simulink model "SWC_FDC_type"  (R2021b)
settings: Solver=FixedStepDiscrete  StartTime=0.0  StopTime=10.0  FixedStep=0.001  RelTol=1e-3
values from neighbouring files (symbols this model uses):
  C_TASK_5MS_S = (	C_TICK_TIME_S      	)    [vcu_local_hdr.m]
  DID_VCUKey = uint16(0x0202)    [vcu_local_hdr.m]
  DID_XWD = uint16(513)    [vcu_local_hdr.m]
  DIDLen_DKCKey = uint16(8)    [vcu_local_hdr.m]
  DIDLen_FoxPiBattSta = uint16(4)    [vcu_local_hdr.m]
  DIDLen_FoxPiBrakeSta = uint16(13)    [vcu_local_hdr.m]
  DIDLen_FoxPiButtonSta = uint16(2)    [vcu_local_hdr.m]
  DIDLen_FoxPiCtrlEnSw = uint16(1)    [vcu_local_hdr.m]
  DIDLen_FoxPiDrivingCtrl = uint16(21)    [vcu_local_hdr.m]
  DIDLen_FoxPiEPSSta = uint16(11)    [vcu_local_hdr.m]
  DIDLen_FoxPiLampCtrl = uint16(6)    [vcu_local_hdr.m]
  DIDLen_FoxPiLampSta = uint16(2)    [vcu_local_hdr.m]
  DIDLen_FoxPiMotionSta = uint16(13)    [vcu_local_hdr.m]
  DIDLen_FoxPiMotorSta = uint16(11)    [vcu_local_hdr.m]
  DIDLen_FoxPiPedalPos = uint16(3)    [vcu_local_hdr.m]
  DIDLen_FoxPiPTGUSSSw = uint16(1)    [vcu_local_hdr.m]
  DIDLen_FoxPiShifterAllow = uint16(3)    [vcu_local_hdr.m]
  DIDLen_FoxPiSwSta = uint16(2)    [vcu_local_hdr.m]
  DIDLen_FoxPiTPMSSta = uint16(13)    [vcu_local_hdr.m]
  DIDLen_FoxPiUSSDist = uint16(20)    [vcu_local_hdr.m]
  DIDLen_FoxPiUSSFaultSta = uint16(2)    [vcu_local_hdr.m]
  DIDLen_FoxPiWheelSpd = uint16(16)    [vcu_local_hdr.m]
  DIDNum_DKCKey = uint16(0x0202)    [vcu_local_hdr.m]
  DIDNum_FoxPiBattSta = uint16(0x100D)    [vcu_local_hdr.m]
  DIDNum_FoxPiBrakeSta = uint16(0x1003)    [vcu_local_hdr.m]
  DIDNum_FoxPiButtonSta = uint16(0x1006)    [vcu_local_hdr.m]
  DIDNum_FoxPiCtrlEnSw = uint16(0x1012)    [vcu_local_hdr.m]
  DIDNum_FoxPiDrivingCtrl = uint16(0x1001)    [vcu_local_hdr.m]
  DIDNum_FoxPiEPSSta = uint16(0x1005)    [vcu_local_hdr.m]
  DIDNum_FoxPiLampCtrl = uint16(0x100C)    [vcu_local_hdr.m]
  DIDNum_FoxPiLampSta = uint16(0x100B)    [vcu_local_hdr.m]
  DIDNum_FoxPiMotionSta = uint16(0x1002)    [vcu_local_hdr.m]
  DIDNum_FoxPiMotorSta = uint16(0x1010)    [vcu_local_hdr.m]
  DIDNum_FoxPiPedalPos = uint16(0x100F)    [vcu_local_hdr.m]
  DIDNum_FoxPiPTGUSSSw = uint16(0x1009)    [vcu_local_hdr.m]
  DIDNum_FoxPiShifterAllow = uint16(0x1011)    [vcu_local_hdr.m]
  DIDNum_FoxPiSwSta = uint16(0x100A)    [vcu_local_hdr.m]
  DIDNum_FoxPiTPMSSta = uint16(0x100E)    [vcu_local_hdr.m]
  DIDNum_FoxPiUSSDist = uint16(0x1007)    [vcu_local_hdr.m]
  DIDNum_FoxPiUSSFaultSta = uint16(0x1008)    [vcu_local_hdr.m]
  DIDNum_FoxPiWheelSpd = uint16(0x1004)    [vcu_local_hdr.m]
  DIDVCUKeyLength = uint16(8)    [vcu_local_hdr.m]
  DTC_10020B = Simulink.Parameter    [DTC_Constant_Definition.m]
  DTC_10020C = Simulink.Parameter    [DTC_Constant_Definition.m]
  DTC_10020D = Simulink.Parameter    [DTC_Constant_Definition.m]
  DTC_10020E = Simulink.Parameter    [DTC_Constant_Definition.m]
  DTC_100210 = Simulink.Parameter    [DTC_Constant_Definition.m]
  DTC_100211 = Simulink.Parameter    [DTC_Constant_Definition.m]
  DTC_100212 = Simulink.Parameter    [DTC_Constant_Definition.m]
  DTC_100213 = Simulink.Parameter    [DTC_Constant_Definition.m]
  DTC_100214 = Simulink.Parameter    [DTC_Constant_Definition.m]
  DTC_100215 = Simulink.Parameter    [DTC_Constant_Definition.m]
  DTC_100216 = Simulink.Parameter    [DTC_Constant_Definition.m]
  DTC_100217 = Simulink.Parameter    [DTC_Constant_Definition.m]
  DTC_100218 = Simulink.Parameter    [DTC_Constant_Definition.m]
  DTC_100219 = Simulink.Parameter    [DTC_Constant_Definition.m]
  DTC_10021A = Simulink.Parameter    [DTC_Constant_Definition.m]
  DTC_10021B = Simulink.Parameter    [DTC_Constant_Definition.m]
  DTC_10021C = Simulink.Parameter    [DTC_Constant_Definition.m]
  DTC_10021D = Simulink.Parameter    [DTC_Constant_Definition.m]
  DTC_10021E = Simulink.Parameter    [DTC_Constant_Definition.m]
  DTC_100220 = Simulink.Parameter    [DTC_Constant_Definition.m]
  DTC_100221 = Simulink.Parameter    [DTC_Constant_Definition.m]
  DTC_100223 = Simulink.Parameter    [DTC_Constant_Definition.m]
  DTC_100224 = Simulink.Parameter    [DTC_Constant_Definition.m]
  DTC_100225 = Simulink.Parameter    [DTC_Constant_Definition.m]
  DTC_100226 = Simulink.Parameter    [DTC_Constant_Definition.m]
  DTC_100227 = Simulink.Parameter    [DTC_Constant_Definition.m]
  DTC_100242 = Simulink.Parameter    [DTC_Constant_Definition.m]
  DTC_100243 = Simulink.Parameter    [DTC_Constant_Definition.m]
  DTC_100244 = Simulink.Parameter    [DTC_Constant_Definition.m]
  DTC_100247 = Simulink.Parameter    [DTC_Constant_Definition.m]
  DTC_100248 = Simulink.Parameter    [DTC_Constant_Definition.m]
  DTC_100249 = Simulink.Parameter    [DTC_Constant_Definition.m]
  DTC_100250 = Simulink.Parameter    [DTC_Constant_Definition.m]
  DTC_100251 = Simulink.Parameter    [DTC_Constant_Definition.m]
  DTC_100252 = Simulink.Parameter    [DTC_Constant_Definition.m]
  DTC_100A10 = Simulink.Parameter    [DTC_Constant_Definition.m]
  DTC_100A12 = Simulink.Parameter    [DTC_Constant_Definition.m]
  DTC_100A16 = Simulink.Parameter    [DTC_Constant_Definition.m]
  DTC_100A17 = Simulink.Parameter    [DTC_Constant_Definition.m]
  DTC_100A18 = Simulink.Parameter    [DTC_Constant_Definition.m]
  DTC_100A19 = Simulink.Parameter    [DTC_Constant_Definition.m]
  DTC_500B01 = Simulink.Parameter    [DTC_Constant_Definition.m]
  DTC_500B02 = Simulink.Parameter    [DTC_Constant_Definition.m]
  DTC_500B03 = Simulink.Parameter    [DTC_Constant_Definition.m]
  DTC_500B04 = Simulink.Parameter    [DTC_Constant_Definition.m]
  DTC_500B05 = Simulink.Parameter    [DTC_Constant_Definition.m]
  DTC_500B06 = Simulink.Parameter    [DTC_Constant_Definition.m]
  DTC_500B07 = Simulink.Parameter    [DTC_Constant_Definition.m]
  DTC_500B08 = Simulink.Parameter    [DTC_Constant_Definition.m]
  DTC_500B09 = Simulink.Parameter    [DTC_Constant_Definition.m]
  DTC_500B0A = Simulink.Parameter    [DTC_Constant_Definition.m]
  DTC_500B0B = Simulink.Parameter    [DTC_Constant_Definition.m]
  DTC_500B0C = Simulink.Parameter    [DTC_Constant_Definition.m]
  DTC_500B0D = Simulink.Parameter    [DTC_Constant_Definition.m]
  DTC_500B0E = Simulink.Parameter    [DTC_Constant_Definition.m]
  DTC_500B0F = Simulink.Parameter    [DTC_Constant_Definition.m]
  DTC_500B10 = Simulink.Parameter    [DTC_Constant_Definition.m]
  DTC_90021F = Simulink.Parameter    [DTC_Constant_Definition.m]
  DTC_90022F = Simulink.Parameter    [DTC_Constant_Definition.m]
  DTC_900253 = Simulink.Parameter    [DTC_Constant_Definition.m]
  DTC_900254 = Simulink.Parameter    [DTC_Constant_Definition.m]
  DTC_900301 = Simulink.Parameter    [DTC_Constant_Definition.m]
  DTC_900302 = Simulink.Parameter    [DTC_Constant_Definition.m]
  DTC_900303 = Simulink.Parameter    [DTC_Constant_Definition.m]
  DTC_900304 = Simulink.Parameter    [DTC_Constant_Definition.m]
  DTC_900305 = Simulink.Parameter    [DTC_Constant_Definition.m]
  DTC_900909 = Simulink.Parameter    [DTC_Constant_Definition.m]
  DTC_90090A = Simulink.Parameter    [DTC_Constant_Definition.m]
  DTC_90090B = Simulink.Parameter    [DTC_Constant_Definition.m]
  DTC_90090C = Simulink.Parameter    [DTC_Constant_Definition.m]
  DTC_90090D = Simulink.Parameter    [DTC_Constant_Definition.m]
  DTC_90090E = Simulink.Parameter    [DTC_Constant_Definition.m]
  DTC_90090F = Simulink.Parameter    [DTC_Constant_Definition.m]
  DTC_900910 = Simulink.Parameter    [DTC_Constant_Definition.m]
  DTC_900911 = Simulink.Parameter    [DTC_Constant_Definition.m]
  DTC_900912 = Simulink.Parameter    [DTC_Constant_Definition.m]
  DTC_900913 = Simulink.Parameter    [DTC_Constant_Definition.m]
  DTC_900914 = Simulink.Parameter    [DTC_Constant_Definition.m]
  ... (+54 more)
undefined symbols (not defined in the file or in its folder): f32_ApsOutVehSpdSig, KHAL_CANBusOffDebounce_cnt, KHAL_CANBusOffDebounce_s, KHAL_DKCDecryptEnable_flg_ovrdflg, KHAL_DKCDecryptEnable_flg_ovrdval, KHAL_RandomNumberY1_enum, KHAL_RandomNumberY2_enum, KHAL_RandomNumberY_ovrdflg, KHAL_TPMSRESBUTT_flg_ovrdflg, KHAL_TPMSRESBUTT_flg_ovrdval, KINP_ReadVinCode_flg, P_boolean, R_DIDWriteCDD_CSOP_DIDSet_DKCKey, R_DIDWriteCDD_CSOP_DIDSet_FoxPiBattSta, R_DIDWriteCDD_CSOP_DIDSet_FoxPiBrakeSta, R_DIDWriteCDD_CSOP_DIDSet_FoxPiButtonSta, R_DIDWriteCDD_CSOP_DIDSet_FoxPiCtrlEnSw, R_DIDWriteCDD_CSOP_DIDSet_FoxPiDrivingCtrl, R_DIDWriteCDD_CSOP_DIDSet_FoxPiEPSSta, R_DIDWriteCDD_CSOP_DIDSet_FoxPiLampCtrl, R_DIDWriteCDD_CSOP_DIDSet_FoxPiLampSta, R_DIDWriteCDD_CSOP_DIDSet_FoxPiMotionSta, R_DIDWriteCDD_CSOP_DIDSet_FoxPiMotorSta, R_DIDWriteCDD_CSOP_DIDSet_FoxPiPedalPos, R_DIDWriteCDD_CSOP_DIDSet_FoxPiPTGUSSSw, R_DIDWriteCDD_CSOP_DIDSet_FoxPiShifterAllow, R_DIDWriteCDD_CSOP_DIDSet_FoxPiSwSta, R_DIDWriteCDD_CSOP_DIDSet_FoxPiTPMSSta, R_DIDWriteCDD_CSOP_DIDSet_FoxPiUSSDist, R_DIDWriteCDD_CSOP_DIDSet_FoxPiUSSFaultSta, R_DIDWriteCDD_CSOP_DIDSet_FoxPiWheelSpd, R_E2E_CAN3_VCU1_CSOP_Write_CAN3_VCU1, R_E2E_CAN3_VCU1_toNIDEC_CSOP_Write_CAN3_VCU1_toNIDEC, R_E2E_CAN4_VCU1_CSOP_Write_CAN4_VCU1, R_FDCCDD_Inner_CSOP_FDC_AppCallSleep, R_HALIN_IMU_CSOP_IMUSetSta, R_HALINCDD_CSOP_PAS_Handler, R_HALINCDD_CSOP_ResetPedalZeroPosDone, R_HALINCDD_CSOP_TPMSSensorIDRegSetResults, R_HALINCDD_CSOP_UDS_Main, R_HALOUT_APS_CSOP_ApsOutput, R_HALOUTCDD_CSOP_AppNmStateReq, R_HALOUTCDD_CSOP_IVIReset, R_HALOUTCDD_CSOP_SetAcoreRebootCmdACK, R_HALOUTCDD_CSOP_SetSysPwrStat ... (+80)
libraries: FVT_lib x447, simulink x289, hcu_lib x19, hdlsllib x9, app x1, halin x1, halout x1, matrix_library x1, inp x1, outp x1
(part 9 of 15)

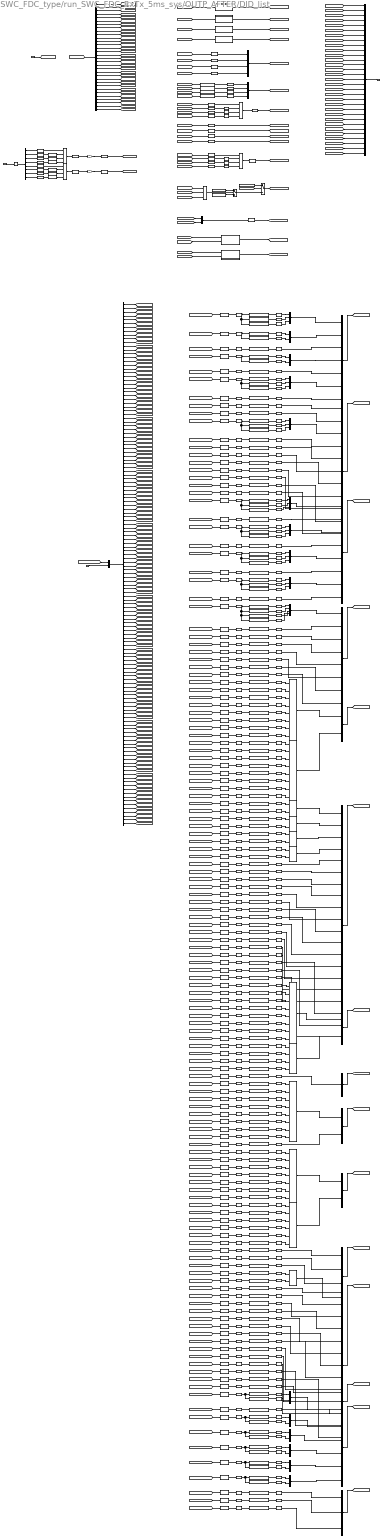
== system SWC_FDC_type/run_SWC_FDC_RxTx_5ms_sys/OUTP_AFTER/DID_list ==
  BOUTP_outputs : Inport
  VHAL_NvmReadArray_raw : Inport  Port=2
  BINP_CANx_outputs : Inport  Port=3
  Bit Shift : hdlsllib/Logic and Bit Operations/Bit Shift  mode=Shift Left Logical  N=3
  Bit Shift1 : hdlsllib/Logic and Bit Operations/Bit Shift  mode=Shift Left Logical  N=2
  Bit Shift2 : hdlsllib/Logic and Bit Operations/Bit Shift  mode=Shift Left Logical  N=1
  Bit Shift3 : hdlsllib/Logic and Bit Operations/Bit Shift  mode=Shift Left Logical  N=3
  Bit Shift4 : hdlsllib/Logic and Bit Operations/Bit Shift  mode=Shift Left Logical  N=2
  Bit Shift5 : hdlsllib/Logic and Bit Operations/Bit Shift  mode=Shift Left Logical  N=1
  Bitwise OR : simulink/Logic and Bit Operations/Bitwise Operator  logicop=OR  UseBitMask=off  NumInputPorts=4  BitMask=bin2dec('11011001')  BitMaskRealWorld=Stored Integer
  Bitwise OR1 : simulink/Logic and Bit Operations/Bitwise Operator  logicop=OR  UseBitMask=off  NumInputPorts=4  BitMask=bin2dec('11011001')  BitMaskRealWorld=Stored Integer
  Bitwise OR13 : simulink/Logic and Bit Operations/Bitwise Operator  logicop=OR  UseBitMask=off  NumInputPorts=4  BitMask=bin2dec('00000000000000000000')  BitMaskRealWorld=Stored Integer
  Bitwise OR14 : simulink/Logic and Bit Operations/Bitwise Operator  logicop=OR  UseBitMask=off  NumInputPorts=4  BitMask=bin2dec('00000000000000000000')  BitMaskRealWorld=Stored Integer
  BitwiseAND{,1,6,8} (4 alike) : simulink/Logic and Bit Operations/Bitwise Operator  logicop=OR  UseBitMask=off  NumInputPorts=8  BitMask=bin2dec('11011001')  BitMaskRealWorld=Stored Integer
  BitwiseAND10 : simulink/Logic and Bit Operations/Bitwise Operator  logicop=OR  UseBitMask=off  NumInputPorts=6  BitMask=bin2dec('11011001')  BitMaskRealWorld=Stored Integer
  BitwiseAND{2..5,11} (5 alike) : simulink/Logic and Bit Operations/Bitwise Operator  logicop=OR  UseBitMask=off  NumInputPorts=2  BitMask=bin2dec('11011001')  BitMaskRealWorld=Stored Integer
  BitwiseAND7 : simulink/Logic and Bit Operations/Bitwise Operator  logicop=OR  UseBitMask=off  NumInputPorts=4  BitMask=bin2dec('11011001')  BitMaskRealWorld=Stored Integer
  BitwiseAND9 : simulink/Logic and Bit Operations/Bitwise Operator  logicop=OR  UseBitMask=off  NumInputPorts=7  BitMask=bin2dec('11011001')  BitMaskRealWorld=Stored Integer
  Bus Creator : BusCreator  Inputs=31
  Bus Creator1 : BusCreator  Inputs=2
  Bus Selector : BusSelector  OutputSignals=VOUTP_WriteChkLFID_raw,VOUTP_WriteChkRFID_raw,VOUTP_WriteChkLRID_raw,VOUTP_WriteChkRRID_raw,VOUTP_LFWheelPress_raw8,VOUTP_RFWheelPress_raw8,VOUTP_LRWheelPress_raw8,VOUTP_RRWheelPress_raw8,VOUTP_LFWheelTemp_C,VOUTP_RFWheelTemp_C,VOUTP_LRWheelTemp_C,VOUTP_RRWheelTemp_C,VOUTP_LFBatWarn_flg,VOUTP_RFBatWarn_flg,VOUTP_LRBatWarn_flg,VOUTP_RRBatWarn_flg,VOUTP_LFWheelPSW_raw8,VOUTP_LRWheelPSW_raw8,VOUTP_RFWheelPSW_raw8,VOUTP_RRWheelPSW_raw8,VOUTP_LFSensorMode_flg,VOUTP_RFSensorMode_flg,VOUTP_LRSensorMode_flg,VOUTP_RRSensorMode_flg,VOUTP_ALFin_flg,VOUTP_ChkStorge_flg,VOUTP_TPMSStorge_flg,VOUTP_unlearnSfali_flg,VOUTP_WritingCnt_enum,VOUTP_LProgress_enum,VOUTP_EAPS1MIN_pct,VOUTP_EAPS2MIN_pct
  Constant : Constant  Value=ENUM_TPMSLearnStatus_LEARNFAIL
  Constant1 : Constant  Value=ENUM_TPMSLearnStatus_NOTLEARN
  Constant2 : Constant  Value=ENUM_TPMSLearnStatus_LEARNED
  Data Type Conversion{1..23} (23 alike) : DataTypeConversion  OutDataTypeStr=uint8
  Data Type Conversion168 : DataTypeConversion  OutDataTypeStr=single
  Data Type Conversion{169..178} (10 alike) : DataTypeConversion  OutDataTypeStr=uint32
  Data Type Conversion179 : DataTypeConversion  OutDataTypeStr=single
  Demux : Demux  Outputs=8
  Logical Operator1 : Logic  Operator=OR  Inputs=3  AllPortsSameDT=off  OutDataTypeStr=boolean
  Multiply1 : Gain  Gain=1/10000
  Multiply2 : Gain  Gain=1/10000
  Mux{,2,12,20} (4 alike) : Mux
  Mux{1,4..5,14,16,18..19,22..28} (14 alike) : Mux  Inputs=2
  Mux{3,6,8,10,30..33} (8 alike) : Mux  Inputs=3
  Mux11 : Mux  Inputs=8
  Mux13 : Mux  Inputs=8
  Mux15 : Mux  Inputs=20
  Mux17 : Mux  Inputs=1
  Mux21 : Mux  Inputs=13
  Mux29 : Mux  Inputs=6
  Mux7 : Mux  Inputs=7
  Mux9 : Mux  Inputs=11
  Selector1 : Selector  InputPortWidth=256  IndexOptions=Index vector (dialog)  Indices=[112:119]  OutputSizes=1
  Shift Arithmetic37 : ArithShift  BitShiftNumber=8  BitShiftDirection=Left
  Shift Arithmetic38 : ArithShift  BitShiftNumber=16  BitShiftDirection=Left
  Shift Arithmetic39 : ArithShift  BitShiftNumber=24  BitShiftDirection=Left
  Shift Arithmetic40 : ArithShift  BitShiftNumber=8  BitShiftDirection=Left
  Shift Arithmetic41 : ArithShift  BitShiftNumber=16  BitShiftDirection=Left
  Shift Arithmetic42 : ArithShift  BitShiftNumber=24  BitShiftDirection=Left
  SignalPack{,9,15,26,30,34,38,43} (8 alike) : FVT_lib/hal/SignalPack_shiftAfterMask  RightShiftCnt=16  BitMask=16711680  LeftShiftCnt=0
  SignalPack{1,3,6,10,16,27,31,35,39,44,147,150,152,154,156,158} (16 alike) : FVT_lib/hal/SignalPack_shiftAfterMask  RightShiftCnt=8  BitMask=65280  LeftShiftCnt=0
  SignalPack{60,68,100,113,121,132} (6 alike) : FVT_lib/hal/SignalPack_shiftAfterMask  RightShiftCnt=0  BitMask=2^1-1  LeftShiftCnt=7
  SignalPack{53,61,92..93,101,105..106,114,122} (9 alike) : FVT_lib/hal/SignalPack_shiftAfterMask  RightShiftCnt=0  BitMask=2^1-1  LeftShiftCnt=0
  SignalPack{54,62,94,102,107,123} (6 alike) : FVT_lib/hal/SignalPack_shiftAfterMask  RightShiftCnt=0  BitMask=2^1-1  LeftShiftCnt=1
  SignalPack{55,63,95,103,108,116,124} (7 alike) : FVT_lib/hal/SignalPack_shiftAfterMask  RightShiftCnt=0  BitMask=2^1-1  LeftShiftCnt=2
  SignalPack{56,64,96,104,109,117,125} (7 alike) : FVT_lib/hal/SignalPack_shiftAfterMask  RightShiftCnt=0  BitMask=2^1-1  LeftShiftCnt=3
  SignalPack{2,4,7,11,17,28,32,36,40,45,148,151,153,155,157,159} (16 alike) : FVT_lib/hal/SignalPack_shiftAfterMask  RightShiftCnt=0  BitMask=255  LeftShiftCnt=0
  SignalPack{57,65,97,110,118,126} (6 alike) : FVT_lib/hal/SignalPack_shiftAfterMask  RightShiftCnt=0  BitMask=2^1-1  LeftShiftCnt=4
  SignalPack{58,66,98,111,119,127} (6 alike) : FVT_lib/hal/SignalPack_shiftAfterMask  RightShiftCnt=0  BitMask=2^1-1  LeftShiftCnt=5
  SignalPack{59,67,99,112,120,131} (6 alike) : FVT_lib/hal/SignalPack_shiftAfterMask  RightShiftCnt=0  BitMask=2^1-1  LeftShiftCnt=6
  SignalPack115 : FVT_lib/hal/SignalPack_shiftAfterMask  RightShiftCnt=0  BitMask=2^2-1  LeftShiftCnt=0
  SignalPack{5,8,12..14,18..25,29,33,37,41,46..52,77..88,128..130,133..144,146,149,160..162} (56 alike) : FVT_lib/hal/SignalPack_shiftAfterMask  RightShiftCnt=0  BitMask=2^8-1  LeftShiftCnt=0
  SignalPack145 : FVT_lib/hal/SignalPack_shiftAfterMask  RightShiftCnt=0  BitMask=2^2-1  LeftShiftCnt=0
  SignalPack42 : FVT_lib/hal/SignalPack_shiftAfterMask  RightShiftCnt=24  BitMask=4278190080  LeftShiftCnt=0
  SignalPack{69,71,73,75,90} (5 alike) : FVT_lib/hal/SignalPack_shiftAfterMask  RightShiftCnt=0  BitMask=2^4-1  LeftShiftCnt=0
  SignalPack{70,72,74,76} (4 alike) : FVT_lib/hal/SignalPack_shiftAfterMask  RightShiftCnt=0  BitMask=2^4-1  LeftShiftCnt=4
  SignalPack89 : FVT_lib/hal/SignalPack_shiftAfterMask  RightShiftCnt=0  BitMask=2^3-1  LeftShiftCnt=0
  SignalPack91 : FVT_lib/hal/SignalPack_shiftAfterMask  RightShiftCnt=0  BitMask=2^2-1  LeftShiftCnt=0
  Switch : Switch  Criteria=u2 ~= 0
  Switch1 : Switch  Criteria=u2 ~= 0
  UnitConverter{,14,24,44,50,56,62,68} (8 alike) : DataTypeConversion  OutDataTypeStr=uint32
  UnitConverter{1..3,5..8,10..13,15..23,25..43,45..49,51..55,57..61,63..67,69..274,276..279,281..282,284..285,287..288,290..291,293..300} (285 alike) : DataTypeConversion  OutDataTypeStr=uint8
  UnitConverter{4,9,275,280,283,286,289,292} (8 alike) : DataTypeConversion  OutDataTypeStr=uint16
  bus_selector : BusSelector  OutputSignals=BINP_CANx_outputs.BINP_CAN1_outputs.VINP_VehSpeed_kph,BINP_CANx_outputs.BINP_CAN1_outputs.VINP_LongAccel_Gps,BINP_CANx_outputs.BINP_CAN1_outputs.VINP_LongAccelV_flg,BINP_CANx_outputs.BINP_CAN1_outputs.VINP_LatAccel_Gps,BINP_CANx_outputs.BINP_CAN1_outputs.VINP_LatAccelV_flg,BINP_CANx_outputs.BINP_CAN1_outputs.VINP_YawRate_degps,BINP_CANx_outputs.BINP_CAN1_outputs.VINP_YawRateV_flg,BINP_CANx_outputs.BINP_CAN1_outputs.VINP_BrkSwSta_flg,BINP_CANx_outputs.BINP_CAN1_outputs.VINP_BrkSwV_flg,BINP_CANx_outputs.BINP_CAN1_outputs.VINP_MCPressure_bar,BINP_CANx_outputs.BINP_CAN1_outputs.VINP_MCPressureV_flg,BINP_CANx_outputs.BINP_CAN1_outputs.VINP_PBAActive_flg,BINP_CANx_outputs.BINP_CAN1_outputs.VINP_PBAFailed_flg,BINP_CANx_outputs.BINP_CAN1_outputs.VINP_ABSActive_flg,BINP_CANx_outputs.BINP_CAN1_outputs.VINP_ABSFailed_flg,BINP_CANx_outputs.BINP_CAN1_outputs.VINP_EBDActive_flg,BINP_CANx_outputs.BINP_CAN1_outputs.VINP_EBDFailed_flg,BINP_CANx_outputs.BINP_CAN1_outputs.VINP_ACCAvail_flg,BINP_CANx_outputs.BINP_CAN1_outputs.VINP_RRRawWhlSpeed_kph,BINP_CANx_outputs.BINP_CAN1_outputs.VINP_RRRawWhlSpeedV_flg,BINP_CANx_outputs.BINP_CAN1_outputs.VINP_LRRawWhlSpeed_kph,BINP_CANx_outputs.BINP_CAN1_outputs.VINP_LRRawWhlSpeedV_flg,BINP_CANx_outputs.BINP_CAN1_outputs.VINP_RFRawWhlSpeed_kph,BINP_CANx_outputs.BINP_CAN1_outputs.VINP_RFRawWhlSpeedV_flg,BINP_CANx_outputs.BINP_CAN1_outputs.VINP_LFRawWhlSpeed_kph,BINP_CANx_outputs.BINP_CAN1_outputs.VINP_LFRawWhlSpeedV_flg,BINP_CANx_outputs.BINP_CAN1_outputs.VINP_SASAngle_Deg,BINP_CANx_outputs.BINP_CAN1_outputs.VINP_SASV_flg,BINP_CANx_outputs.BINP_CAN1_outputs.VINP_SASCAL_flg,BINP_CANx_outputs.BINP_CAN1_outputs.VINP_EPSAOIControl_enum,BINP_CANx_outputs.BINP_CAN1_outputs.VINP_EpasFailed_enum,BINP_CANx_outputs.BINP_CAN1_outputs.VINP_EPSTOIActivation_flg,BINP_CANx_outputs.BINP_CAN1_outputs.VINP_EPSTOIUnavailable_flg,BINP_CANx_outputs.BINP_CAN1_outputs.VINP_EPSTOIFault_flg,BINP_CANx_outputs.BINP_CAN4_outputs.VINP_SWCACCSta_flg,BINP_CANx_outputs.BINP_CAN4_outputs.VINP_SWCCANCELSta_flg,BINP_CANx_outputs.BINP_CAN4_outputs.VINP_SWCSetdownSta_flg,BINP_CANx_outputs.BINP_CAN4_outputs.VINP_SWCResUpSta_flg,BINP_CANx_outputs.BINP_CAN4_outputs.VINP_SWCDistanceSta_flg,BINP_CANx_outputs.BINP_CAN4_outputs.VINP_SWCmodeSta_flg,BINP_CANx_outputs.BINP_CAN4_outputs.VINP_SWCUpSta_flg,BINP_CANx_outputs.BINP_CAN4_outputs.VINP_SWCDownSta_flg,BINP_CANx_outputs.BINP_CAN4_outputs.VINP_SWCLeftSta_flg,BINP_CANx_outputs.BINP_CAN4_outputs.VINP_SWCRightSta_flg,BINP_CANx_outputs.BINP_CAN4_outputs.VINP_SWCRegenDown_flg,BINP_CANx_outputs.BINP_CAN4_outputs.VINP_SWCUndefinedSta_flg,BINP_CANx_outputs.BINP_CAN4_outputs.VINP_SWCVRSta_flg,BINP_CANx_outputs.BINP_CAN4_outputs.VINP_SWCLKASta_flg,BINP_CANx_outputs.BINP_CAN4_outputs.VINP_SWCRegenUp_flg,BINP_CANx_outputs.BINP_CAN4_outputs.VINP_SWCTripSta_flg,BOUTP_outputs.VOUTP_PASARMR_enum,BOUTP_outputs.VOUTP_PASARML_enum,BOUTP_outputs.VOUTP_PASARCR_enum,BOUTP_outputs.VOUTP_PASARCL_enum,BOUTP_outputs.VOUTP_PASAFMR_enum,BOUTP_outputs.VOUTP_PASAFML_enum,BOUTP_outputs.VOUTP_PASAFCR_enum,BOUTP_outputs.VOUTP_PASAFCL_enum,BOUTP_outputs.VOUTP_PASDRMR_cm,BOUTP_outputs.VOUTP_PASDRML_cm,BOUTP_outputs.VOUTP_PASDRCR_cm,BOUTP_outputs.VOUTP_PASDRCL_cm,BOUTP_outputs.VOUTP_PASDFMR_cm,BOUTP_outputs.VOUTP_PASDFML_cm,BOUTP_outputs.VOUTP_PASDFCR_cm,BOUTP_outputs.VOUTP_PASDFCL_cm,BOUTP_outputs.VOUTP_APSDFLL_cm,BOUTP_outputs.VOUTP_APSDFLR_cm,BOUTP_outputs.VOUTP_APSDRLL_cm,BOUTP_outputs.VOUTP_APSDRLR_cm,BOUTP_outputs.VOUTP_Chime_enum,BOUTP_outputs.VOUTP_SNSRLayout_enum,BOUTP_outputs.VOUTP_ModOperation_enum,BOUTP_outputs.VOUTP_StaFSya_flg,BOUTP_outputs.VOUTP_USSStaRMR_flg,BOUTP_outputs.VOUTP_USSStaRML_flg,BOUTP_outputs.VOUTP_USSStaRCR_flg,BOUTP_outputs.VOUTP_USSStaRCL_flg,BOUTP_outputs.VOUTP_USSStaFMR_flg,BOUTP_outputs.VOUTP_USSStaFML_flg,BOUTP_outputs.VOUTP_USSStaFCR_flg,BOUTP_outputs.VOUTP_USSStaFCL_flg,BOUTP_outputs.VOUTP_USSStaRLR_flg,BOUTP_outputs.VOUTP_USSStaRLL_flg,BOUTP_outputs.VOUTP_USSStaFLR_flg,BOUTP_outputs.VOUTP_USSStaFLL_flg,BINP_CANx_outputs.BINP_CAN2_outputs.VINP_IVIPTGUSStaSW_flg,BOUTP_outputs.VOUTP_CrashDetd_flg,BINP_CANx_outputs.BINP_CAN4_outputs.VINP_DrLockSta_flg,BOUTP_outputs.VOUTP_AllDoorSW_flg,BOUTP_outputs.VOUTP_DrDoorSW_flg,BOUTP_outputs.VOUTP_PsDoorSW_flg,BOUTP_outputs.VOUTP_RLDoorSW_flg,BOUTP_outputs.VOUTP_RRDoorSW_flg,BOUTP_outputs.VOUTP_TailgateSW_flg,BOUTP_outputs.VOUTP_HoodSW_flg,BOUTP_outputs.VOUTP_TurnSwSta_enum,BOUTP_outputs.VOUTP_DimSwSta_flg,BOUTP_outputs.VOUTP_PassSWSta_flg,BOUTP_outputs.VOUTP_PosLamp_flg,BOUTP_outputs.VOUTP_LBeam_flg,BOUTP_outputs.VOUTP_HBeam_flg,BOUTP_outputs.VOUTP_RDRL_flg,BOUTP_outputs.VOUTP_LDRL_flg,BOUTP_outputs.VOUTP_LTurnLP_flg,BOUTP_outputs.VOUTP_RTurnLP_flg,BOUTP_outputs.VOUTP_BrakeLamp_flg,BOUTP_outputs.VOUTP_ReverseLamp_flg,BOUTP_outputs.VOUTP_RrFogLamp_flg,BINP_CANx_outputs.BINP_CAN3_outputs.VINP_LVBattDet12V_V,BINP_CANx_outputs.BINP_CAN3_outputs.VINP_HVBattSOC_pct,BINP_CANx_outputs.BINP_CAN3_outputs.VINP_CellTempAvg_C,BINP_CANx_outputs.BINP_CAN3_outputs.VINP_HVBContactorSta_flg,BINP_CANx_outputs.BINP_CAN3_outputs.VINP_HVBattErr_flg,BOUTP_outputs.VOUTP_LFWheelPress_raw8,BOUTP_outputs.VOUTP_RFWheelPress_raw8,BOUTP_outputs.VOUTP_LRWheelPress_raw8,BOUTP_outputs.VOUTP_RRWheelPress_raw8,BOUTP_outputs.VOUTP_LFWheelTemp_C,BOUTP_outputs.VOUTP_RFWheelTemp_C,BOUTP_outputs.VOUTP_LRWheelTemp_C,BOUTP_outputs.VOUTP_RRWheelTemp_C,BOUTP_outputs.VOUTP_LFWheelPSW_raw8,BOUTP_outputs.VOUTP_RFWheelPSW_raw8,BOUTP_outputs.VOUTP_LRWheelPSW_raw8,BOUTP_outputs.VOUTP_RRWheelPSW_raw8,BOUTP_outputs.VOUTP_TPMSWarnIndi_enum,BOUTP_outputs.VOUTP_ActAPSPosn_pct,BINP_CANx_outputs.BINP_CAN1_outputs.VINP_BrkPedalPos_pct,BOUTP_outputs.VOUTP_TqSourceRr_enum,BOUTP_outputs.VOUTP_RrTMTqReq_Nm,BINP_CANx_outputs.BINP_CAN3_outputs.VINP_RrEDURealTMTqNidec_Nm,BINP_CANx_outputs.BINP_CAN3_outputs.VINP_RrMotorAvailTqNidec_Nm,BINP_CANx_outputs.BINP_CAN3_outputs.VINP_RrRegenAvailTqNidec_Nm,BINP_CANx_outputs.BINP_CAN3_outputs.VINP_RrTMSpdNidec_rpm,BOUTP_outputs.VOUTP_ExternalTqAllow_flg,BOUTP_outputs.VOUTP_ExtShftAllow_flg,BOUTP_outputs.VOUTP_ExtDoorAllow_flg
  convert_out{,1..3,111,118..121} (9 alike) : FVT_lib/hal/convert_out  gain=1  offset=-40
  convert_out{6,8,10..17,19,21,23,25,27..92,94..108,112..113,126,129,135..141} (106 alike) : FVT_lib/hal/convert_out  gain=1  offset=0
  convert_out109 : FVT_lib/hal/convert_out  gain=0.1  offset=0
  convert_out110 : FVT_lib/hal/convert_out  gain=0.4  offset=0
  convert_out{114..117,122..125} (8 alike) : FVT_lib/hal/convert_out  gain=0.25  offset=7.26
  convert_out127 : FVT_lib/hal/convert_out  gain=0.394  offset=0
  convert_out128 : FVT_lib/hal/convert_out  gain=0.4  offset=0
  convert_out130 : FVT_lib/hal/convert_out  gain=1  offset=-530
  convert_out131 : FVT_lib/hal/convert_out  gain=1  offset=-1023
  convert_out132 : FVT_lib/hal/convert_out  gain=1  offset=-1023
  convert_out133 : FVT_lib/hal/convert_out  gain=1  offset=-1023
  convert_out134 : FVT_lib/hal/convert_out  gain=1  offset=-32767
  convert_out{18,20,22,24} (4 alike) : FVT_lib/hal/convert_out  gain=0.0625  offset=0
  convert_out26 : FVT_lib/hal/convert_out  gain=0.1  offset=-900
  convert_out4 : FVT_lib/hal/convert_out  gain=0.125  offset=0
  convert_out5 : FVT_lib/hal/convert_out  gain=0.01  offset=-1.27
  convert_out7 : FVT_lib/hal/convert_out  gain=0.01  offset=-1.27
  convert_out9 : FVT_lib/hal/convert_out  gain=0.1  offset=-100
  convert_out93 : FVT_lib/hal/convert_out  gain=0.1  offset=-9.7
  pct2raw1 : Subsystem
  pct2raw8 : Subsystem
  uint32Touint8Array : Subsystem
  uint32Touint8Array1 : Subsystem
  uint32Touint8Array2 : Subsystem
  uint32Touint8Array3 : Subsystem
  BOUTP_DIDSetData_outputs : Outport
  wires:
  Bus Selector/1 -> [VOUTP_WriteChkLFID_raw]  "<VOUTP_WriteChkLFID_raw>"
  Bus Selector/2 -> [VOUTP_WriteChkRFID_raw]  "<VOUTP_WriteChkRFID_raw>"
  Bus Selector/4 -> [VOUTP_WriteChkRRID_raw]  "<VOUTP_WriteChkRRID_raw>"
  Bus Selector/3 -> [VOUTP_WriteChkLRID_raw]  "<VOUTP_WriteChkLRID_raw>"
  Bus Selector/5 -> [VOUTP_LFWheelPress_raw8]  "<VOUTP_LFWheelPress_raw8>"
  Bus Selector/6 -> [VOUTP_RFWheelPress_raw8]  "<VOUTP_RFWheelPress_raw8>"
  Bus Selector/7 -> [VOUTP_LRWheelPress_raw8]  "<VOUTP_LRWheelPress_raw8>"
  Bus Selector/8 -> [VOUTP_RRWheelPress_raw8]  "<VOUTP_RRWheelPress_raw8>"
  Bus Selector/13 -> [VOUTP_LFBatWarn_flg]  "<VOUTP_LFBatWarn_flg>"
  Bus Selector/14 -> [VOUTP_RFBatWarn_flg]  "<VOUTP_RFBatWarn_flg>"
  Bus Selector/15 -> [VOUTP_LRBatWarn_flg]  "<VOUTP_LRBatWarn_flg>"
  Bus Selector/16 -> [VOUTP_RRBatWarn_flg]  "<VOUTP_RRBatWarn_flg>"
  Bus Selector/18 -> [VOUTP_LRWheelPSW_raw8]  "<VOUTP_LRWheelPSW_raw8>"
  Bus Selector/19 -> [VOUTP_RFWheelPSW_raw8]  "<VOUTP_RFWheelPSW_raw8>"
  Bus Selector/20 -> [VOUTP_RRWheelPSW_raw8]  "<VOUTP_RRWheelPSW_raw8>"
  Bus Selector/17 -> [VOUTP_LFWheelPSW_raw8]  "<VOUTP_LFWheelPSW_raw8>"
  Bus Selector/21 -> [VOUTP_LFSensorMode_flg]  "<VOUTP_LFSensorMode_flg>"
  Bus Selector/22 -> [VOUTP_RFSensorMode_flg]  "<VOUTP_RFSensorMode_flg>"
  Bus Selector/23 -> [VOUTP_LRSensorMode_flg]  "<VOUTP_LRSensorMode_flg>"
  Bus Selector/24 -> [VOUTP_RRSensorMode_flg]  "<VOUTP_RRSensorMode_flg>"
  Bus Selector/27 -> [VOUTP_TPMSStorge_flg]  "<VOUTP_TPMSStorge_flg>"
  Bus Selector/25 -> [VOUTP_ALFin_flg]  "<VOUTP_ALFin_flg>"
  Bus Selector/26 -> [VOUTP_ChkStorge_flg]  "<VOUTP_ChkStorge_flg>"
  Bus Selector/28 -> [VOUTP_unlearnSfali_flg]  "<VOUTP_unlearnSfali_flg>"
  Bus Selector/9 -> [VOUTP_LFWheelTemp_C]  "<VOUTP_LFWheelTemp_C>"
  Bus Selector/10 -> [VOUTP_RFWheelTemp_C]  "<VOUTP_RFWheelTemp_C>"
  Bus Selector/11 -> [VOUTP_LRWheelTemp_C]  "<VOUTP_LRWheelTemp_C>"
  Bus Selector/12 -> [VOUTP_RRWheelTemp_C]  "<VOUTP_RRWheelTemp_C>"
  Data Type Conversion8/1 -> Mux2/1
  Data Type Conversion9/1 -> Mux2/2
  Data Type Conversion10/1 -> Mux2/3
  Data Type Conversion11/1 -> Mux2/4
  [VOUTP_LFWheelPSW_raw8] -> Data Type Conversion6/1
  [VOUTP_RRWheelPSW_raw8] -> Data Type Conversion5/1
  [VOUTP_LFSensorMode_flg] -> Data Type Conversion21/1
  [VOUTP_RRSensorMode_flg] -> Data Type Conversion14/1
  [VOUTP_LRSensorMode_flg] -> Data Type Conversion12/1
  [VOUTP_RFSensorMode_flg] -> Data Type Conversion13/1
  Data Type Conversion21/1 -> Bitwise OR/1
  Data Type Conversion12/1 -> Bit Shift1/1
  Data Type Conversion14/1 -> Bit Shift/1
  Constant1/1 -> Switch1/3
  [VOUTP_ALFin_flg] -> Logical Operator1/1
  Switch1/1 -> Switch/3
  [VOUTP_ChkStorge_flg] -> Logical Operator1/2
  Constant/1 -> Switch/1
  Constant2/1 -> Switch1/1
  [VOUTP_TPMSStorge_flg] -> Logical Operator1/3
  Logical Operator1/1 -> Switch1/2
  [VOUTP_unlearnSfali_flg] -> Switch/2
  Mux/1 -> [VHAL_DIDSetWhlPres_raw8]
  Mux2/1 -> [VHAL_DIDSetWhlTmp_raw8]
  Data Type Conversion6/1 -> [VHAL_DIDSetLFLowPresThre_raw8]
  Data Type Conversion7/1 -> [VHAL_DIDSetRFLowPresThre_raw8]
  Data Type Conversion4/1 -> [VHAL_DIDSetLRLowPresThre_raw8]
  Data Type Conversion5/1 -> [VHAL_DIDSetRRLowPresThre_raw8]
  Bitwise OR/1 -> Data Type Conversion20/1
  Switch/1 -> [VHAL_DIDSetTPMSLearnSta_raw8]
  Bit Shift/1 -> Bitwise OR/4
  Bit Shift1/1 -> Bitwise OR/3
  Bit Shift2/1 -> Bitwise OR/2
  Data Type Conversion20/1 -> [VHAL_DIDSetSensorMode_raw8]
  Data Type Conversion13/1 -> Bit Shift2/1
  [VOUTP_RFBatWarn_flg] -> Data Type Conversion2/1
  Data Type Conversion1/1 -> Bit Shift4/1
  [VOUTP_LRBatWarn_flg] -> Data Type Conversion1/1
  [VOUTP_LFBatWarn_flg] -> Data Type Conversion22/1
  Bitwise OR1/1 -> Data Type Conversion15/1
  Bit Shift4/1 -> Bitwise OR1/3
  Data Type Conversion2/1 -> Bit Shift5/1
  Bit Shift3/1 -> Bitwise OR1/4
  Data Type Conversion22/1 -> Bitwise OR1/1
  Data Type Conversion3/1 -> Bit Shift3/1
  Bit Shift5/1 -> Bitwise OR1/2
  [VOUTP_RRBatWarn_flg] -> Data Type Conversion3/1
  Data Type Conversion15/1 -> [VHAL_DIDSetWhlSensorBattSta_raw8]
  [VHAL_DIDSetTPMSLearnSta_raw8] -> Bus Creator/13  "VHAL_DIDSetTPMSLearnSta_raw8"
  [VHAL_DIDSetLFSensorID_raw8] -> Bus Creator/1  "VHAL_DIDSetLFSensorID_raw8"
  [VHAL_DIDSetRFSensorID_raw8] -> Bus Creator/2  "VHAL_DIDSetRFSensorID_raw8"
  [VHAL_DIDSetLRSensorID_raw8] -> Bus Creator/3  "VHAL_DIDSetLRSensorID_raw8"
  [VHAL_DIDSetRRSensorID_raw8] -> Bus Creator/4  "VHAL_DIDSetRRSensorID_raw8"
  [VHAL_DIDSetWhlPres_raw8] -> Bus Creator/5  "VHAL_DIDSetWhlPres_raw8"
  [VHAL_DIDSetWhlTmp_raw8] -> Bus Creator/6  "VHAL_DIDSetWhlTmp_raw8"
  [VHAL_DIDSetWhlSensorBattSta_raw8] -> Bus Creator/7  "VHAL_DIDSetWhlSensorBattSta_raw8"
  [VHAL_DIDSetLFLowPresThre_raw8] -> Bus Creator/8  "VHAL_DIDSetLFLowPresThre_raw8"
  [VHAL_DIDSetRFLowPresThre_raw8] -> Bus Creator/9  "VHAL_DIDSetRFLowPresThre_raw8"
  [VHAL_DIDSetLRLowPresThre_raw8] -> Bus Creator/10  "VHAL_DIDSetLRLowPresThre_raw8"
  [VHAL_DIDSetRRLowPresThre_raw8] -> Bus Creator/11  "VHAL_DIDSetRRLowPresThre_raw8"
  [VHAL_DIDSetSensorMode_raw8] -> Bus Creator/12  "VHAL_DIDSetSensorMode_raw8"
  Bus Creator/1 -> BOUTP_DIDSetData_outputs/1
  [VOUTP_WriteChkLFID_raw] -> uint32Touint8Array/1(In1)
  uint32Touint8Array/1(Out1) -> [VHAL_DIDSetLFSensorID_raw8]
  [VOUTP_WriteChkRFID_raw] -> uint32Touint8Array1/1(In1)
  uint32Touint8Array1/1(Out1) -> [VHAL_DIDSetRFSensorID_raw8]
  [VOUTP_WriteChkLRID_raw] -> uint32Touint8Array2/1(In1)
  uint32Touint8Array2/1(Out1) -> [VHAL_DIDSetLRSensorID_raw8]
  [VOUTP_WriteChkRRID_raw] -> uint32Touint8Array3/1(In1)
  uint32Touint8Array3/1(Out1) -> [VHAL_DIDSetRRSensorID_raw8]
  [VOUTP_RFWheelPress_raw8] -> Data Type Conversion17/1
  [VOUTP_LFWheelPress_raw8] -> Data Type Conversion16/1
  [VOUTP_LRWheelPress_raw8] -> Data Type Conversion18/1
  [VOUTP_RRWheelPress_raw8] -> Data Type Conversion19/1
  convert_out/1 -> Data Type Conversion8/1
  convert_out1/1 -> Data Type Conversion9/1
  convert_out2/1 -> Data Type Conversion10/1
  convert_out3/1 -> Data Type Conversion11/1
  Data Type Conversion16/1 -> Mux/1
  Data Type Conversion17/1 -> Mux/2
  Data Type Conversion18/1 -> Mux/3
  Data Type Conversion19/1 -> Mux/4
  [VOUTP_LFWheelTemp_C] -> convert_out/1
  [VOUTP_RFWheelTemp_C] -> convert_out1/1
  [VOUTP_LRWheelTemp_C] -> convert_out2/1
  [VOUTP_RRWheelTemp_C] -> convert_out3/1
  [VOUTP_RFWheelPSW_raw8] -> Data Type Conversion7/1
  [VOUTP_LRWheelPSW_raw8] -> Data Type Conversion4/1
  Bus Selector/29 -> [VOUTP_WritingCnt_enum]  "<VOUTP_WritingCnt_enum>"
  Bus Selector/30 -> [VOUTP_LProgress_enum]  "<VOUTP_LProgress_enum>"
  [VOUTP_WritingCnt_enum] -> Mux1/2
  [VHAL_TPMSSensorIDRegResults_raw8] -> Bus Creator/14  "VHAL_TPMSSensorIDRegResults_raw8"
  Data Type Conversion23/1 -> [VHAL_TPMSSensorIDRegResults_raw8]
  [VOUTP_LProgress_enum] -> Mux1/1
  Mux1/1 -> Data Type Conversion23/1
  pct2raw8/1(PedalZP_raw8) -> [VHAL_DIDSetAPPPedalZP_raw8]
  pct2raw1/1(PedalZP_raw8) -> [VHAL_DIDSetNVMPedalZP_raw8]
  [VHAL_DIDSetAPPPedalZP_raw8] -> Bus Creator/15  "VHAL_DIDSetAPPPedalZP_raw8"
  [VHAL_DIDSetNVMPedalZP_raw8] -> Bus Creator/16  "VHAL_DIDSetNVMPedalZP_raw8"
  Data Type Conversion174/1 -> Bitwise OR14/1
  Demux/7 -> Data Type Conversion176/1
  Data Type Conversion170/1 -> Shift Arithmetic37/1
  Demux/2 -> Data Type Conversion170/1
  Data Type Conversion168/1 -> [VHAL_EAPS2MINMem_pct]
  Data Type Conversion172/1 -> Shift Arithmetic39/1
  Data Type Conversion169/1 -> Bitwise OR13/1
  Data Type Conversion175/1 -> Shift Arithmetic40/1
  Data Type Conversion176/1 -> Shift Arithmetic41/1
  Data Type Conversion173/1 -> Multiply1/1
  Data Type Conversion177/1 -> Shift Arithmetic42/1
  Data Type Conversion178/1 -> Multiply2/1
  Multiply2/1 -> Data Type Conversion168/1
  Data Type Conversion171/1 -> Shift Arithmetic38/1
  Demux/8 -> Data Type Conversion177/1
  Demux/5 -> Data Type Conversion174/1
  Demux/6 -> Data Type Conversion175/1
  Bitwise OR13/1 -> Data Type Conversion173/1
  Shift Arithmetic41/1 -> Bitwise OR14/3
  Demux/3 -> Data Type Conversion171/1
  Bitwise OR14/1 -> Data Type Conversion178/1
  Shift Arithmetic39/1 -> Bitwise OR13/4
  Multiply1/1 -> Data Type Conversion179/1
  Shift Arithmetic38/1 -> Bitwise OR13/3
  Demux/4 -> Data Type Conversion172/1
  Data Type Conversion179/1 -> [VHAL_EAPS1MINMem_pct]
  Shift Arithmetic42/1 -> Bitwise OR14/4
  Shift Arithmetic40/1 -> Bitwise OR14/2
  Shift Arithmetic37/1 -> Bitwise OR13/2
  Demux/1 -> Data Type Conversion169/1
  Selector1/1 -> Demux/1
  VHAL_NvmReadArray_raw/1 -> Selector1/1
  Bus Selector/31 -> [VOUTP_EAPS1MIN_pct]  "<VOUTP_EAPS1MIN_pct>"
  Bus Selector/32 -> [VOUTP_EAPS2MIN_pct]  "<VOUTP_EAPS2MIN_pct>"
  [VOUTP_EAPS1MIN_pct] -> pct2raw8/1(EAPS1_pct)
  [VOUTP_EAPS2MIN_pct] -> pct2raw8/2(EAPS2_pct)
  [VHAL_EAPS1MINMem_pct] -> pct2raw1/1(EAPS1_pct)
  [VHAL_EAPS2MINMem_pct] -> pct2raw1/2(EAPS2_pct)
  [FoxPiMotionStatus] -> Bus Creator/17  "VHAL_DIDSetFoxPiMotionSta_raw8"
  [FoxPiBrakeStatus] -> Bus Creator/18  "VHAL_DIDSetFoxPiBrakeSta_raw8"
  [FoxPiWheelSpeed] -> Bus Creator/19  "VHAL_DIDSetFoxPiWheelSpd_raw8"
  [FoxPiEPSStatus] -> Bus Creator/20  "VHAL_DIDSetFoxPiEPSSta_raw8"
  [FoxPiButtonStatus] -> Bus Creator/21  "VHAL_DIDSetFoxPiButtonSta_raw8"
  [FoxPiSwitchStatus] -> Bus Creator/25  "VHAL_DIDSetFoxPiSwSta_raw8"
  [FoxPiPTGUSSSW] -> Bus Creator/24  "VHAL_DIDSetFoxPiPTGUSSSw_raw8"
  [FoxPiUSSFaultStatus] -> Bus Creator/23  "VHAL_DIDSetFoxPiUSSFaultSta_raw8"
  [FoxPiUSSDistance] -> Bus Creator/22  "VHAL_DIDSetFoxPiUSSDist_raw8"
  [FoxPiLampStatus] -> Bus Creator/26  "VHAL_DIDSetFoxPiLampSta_raw8"
  [FoxPiBatteryStatus] -> Bus Creator/27  "VHAL_DIDSetFoxPiBattSta_raw8"
  [FoxPiTPMSStatus] -> Bus Creator/28  "VHAL_DIDSetFoxPiTPMSSta_raw8"
  [FoxPiPedalposition] -> Bus Creator/29  "VHAL_DIDSetFoxPiPedalPos_raw8"
  [FoxPiShifterallow] -> Bus Creator/31  "VHAL_DIDSetFoxPiShifterAllow_raw8"
  [FoxPiMotorStatus] -> Bus Creator/30  "VHAL_DIDSetFoxPiMotorSta_raw8"
  BOUTP_outputs/1 -> [BOUTP_outputs]
  [BOUTP_outputs] -> Bus Selector/1
  ? -> ?
  bus_selector/18 -> [ACCAvailabliity]  "<VINP_ACCAvail_flg>"
  bus_selector/57 -> [PASAFCR]  "<VOUTP_PASAFCR_enum>"
  bus_selector/84 -> [USSStaRLL]  "<VOUTP_USSStaRLL_flg>"
  bus_selector/80 -> [USSStaFML]  "<VOUTP_USSStaFML_flg>"
  bus_selector/52 -> [PASARML]  "<VOUTP_PASARML_enum>"
  bus_selector/65 -> [PASDFCR]  "<VOUTP_PASDFCR_cm>"
  bus_selector/50 -> [SWCTripSta]  "<VINP_SWCTripSta_flg>"
  bus_selector/97 -> [ColumnTurnlampSwitchStatus]  "<VOUTP_TurnSwSta_enum>"
  bus_selector/69 -> [APSDRLL]  "<VOUTP_APSDRLL_cm>"
  bus_selector/85 -> [USSStaFLR]  "<VOUTP_USSStaFLR_flg>"
  bus_selector/81 -> [USSStaFCR]  "<VOUTP_USSStaFCR_flg>"
  bus_selector/79 -> [USSStaFMR]  "<VOUTP_USSStaFMR_flg>"
  bus_selector/126 -> [RightRearLowPressureThreshold]  "<VOUTP_RRWheelPSW_raw8>"
  bus_selector/110 -> [LVBattDet12V]  "<VINP_LVBattDet12V_V>"
  bus_selector/104 -> [LeftDaytimeRunningLightStatus]  "<VOUTP_LDRL_flg>"
  bus_selector/99 -> [ColumnPassSwitchStatus]  "<VOUTP_PassSWSta_flg>"
  bus_selector/71 -> [PASChime]  "<VOUTP_Chime_enum>"
  bus_selector/127 -> [TPMSWarnindi]  "<VOUTP_TPMSWarnIndi_enum>"
  bus_selector/133 -> [RrMotorAvailTq]  "<VINP_RrMotorAvailTqNidec_Nm>"
  bus_selector/122 -> [RightRearWheelTemperature]  "<VOUTP_RRWheelTemp_C>"
  bus_selector/129 -> [BrkPedalPos]  "<VINP_BrkPedalPos_pct>"
  bus_selector/135 -> [TMSpd]  "<VINP_RrTMSpdNidec_rpm>"
  bus_selector/131 -> [RrTMTqReqtoNidec]  "<VOUTP_RrTMTqReq_Nm>"
  bus_selector/20 -> [RRRawWhlSpeedV]  "<VINP_RRRawWhlSpeedV_flg>"
  bus_selector/75 -> [USSStaRMR]  "<VOUTP_USSStaRMR_flg>"
  bus_selector/120 -> [RightForwardWheelTemperature]  "<VOUTP_RFWheelTemp_C>"
  bus_selector/118 -> [RightRearWheelPressure]  "<VOUTP_RRWheelPress_raw8>"
  bus_selector/116 -> [RightForwardWheelPressure]  "<VOUTP_RFWheelPress_raw8>"
  bus_selector/4 -> [LatAccel]  "<VINP_LatAccel_Gps>"
  bus_selector/114 -> [HVBattErr]  "<VINP_HVBattErr_flg>"
  bus_selector/112 -> [CellTempAvg]  "<VINP_CellTempAvg_C>"
  bus_selector/138 -> [VTQDExtDoorAllowflg]  "<VOUTP_ExtDoorAllow_flg>"
  bus_selector/134 -> [RrRegenAvailTq]  "<VINP_RrRegenAvailTqNidec_Nm>"
  bus_selector/132 -> [RrEDURealTMTqNidec]  "<VINP_RrEDURealTMTqNidec_Nm>"
  bus_selector/78 -> [USSStaRCL]  "<VOUTP_USSStaRCL_flg>"
  bus_selector/92 -> [PassengerDoorSwitchStatus]  "<VOUTP_PsDoorSW_flg>"
  bus_selector/48 -> [SWCLKASta]  "<VINP_SWCLKASta_flg>"
  bus_selector/83 -> [USSStaRLR]  "<VOUTP_USSStaRLR_flg>"
  bus_selector/54 -> [PASARCL]  "<VOUTP_PASARCL_enum>"
  bus_selector/47 -> [SWCVRSta]  "<VINP_SWCVRSta_flg>"
  bus_selector/111 -> [HVBattSOC]  "<VINP_HVBattSOC_pct>"
  bus_selector/3 -> [LongAccelV]  "<VINP_LongAccelV_flg>"
  bus_selector/39 -> [SWCDistanceSta]  "<VINP_SWCDistanceSta_flg>"
  bus_selector/19 -> [RRRawWhlSpeed]  "<VINP_RRRawWhlSpeed_kph>"
  bus_selector/9 -> [BrkSwV]  "<VINP_BrkSwV_flg>"
  bus_selector/88 -> [CrashDetectStatus]  "<VOUTP_CrashDetd_flg>"
  bus_selector/38 -> [SWCRESupSta]  "<VINP_SWCResUpSta_flg>"
  bus_selector/29 -> [SASCAL]  "<VINP_SASCAL_flg>"
  bus_selector/119 -> [LeftForwardWheelTemperature]  "<VOUTP_LFWheelTemp_C>"
  bus_selector/89 -> [DriverLockStatus]  "<VINP_DrLockSta_flg>"
  bus_selector/62 -> [PASDRCL]  "<VOUTP_PASDRCL_cm>"
  bus_selector/60 -> [PASDRML]  "<VOUTP_PASDRML_cm>"
  bus_selector/49 -> [SWCRegenUp]  "<VINP_SWCRegenUp_flg>"
  bus_selector/117 -> [LeftRearWheelPressure]  "<VOUTP_LRWheelPress_raw8>"
  bus_selector/123 -> [LeftForwardLowPressureThreshold]  "<VOUTP_LFWheelPSW_raw8>"
  bus_selector/55 -> [PASAFMR]  "<VOUTP_PASAFMR_enum>"
  bus_selector/136 -> [VTQDExternalTqAllowflg]  "<VOUTP_ExternalTqAllow_flg>"
  bus_selector/6 -> [YawRate]  "<VINP_YawRate_degps>"
  bus_selector/86 -> [USSStaFLL]  "<VOUTP_USSStaFLL_flg>"
  bus_selector/74 -> [PASStaFSys]  "<VOUTP_StaFSya_flg>"
  bus_selector/72 -> [PASSNSRLayout]  "<VOUTP_SNSRLayout_enum>"
  bus_selector/56 -> [PASAFML]  "<VOUTP_PASAFML_enum>"
  bus_selector/15 -> [ABSFailed]  "<VINP_ABSFailed_flg>"
  bus_selector/66 -> [PASDFCL]  "<VOUTP_PASDFCL_cm>"
  bus_selector/1 -> [Vehiclespeed]  "<VINP_VehSpeed_kph>"
  bus_selector/68 -> [APSDFLR]  "<VOUTP_APSDFLR_cm>"
  bus_selector/98 -> [ColumnDimSwitchStatus]  "<VOUTP_DimSwSta_flg>"
  bus_selector/103 -> [RightDaytimeRunningLightStatus]  "<VOUTP_RDRL_flg>"
  bus_selector/70 -> [APSDRLR]  "<VOUTP_APSDRLR_cm>"
  bus_selector/64 -> [PASDFML]  "<VOUTP_PASDFML_cm>"
  bus_selector/67 -> [APSDFLL]  "<VOUTP_APSDFLL_cm>"
  bus_selector/87 -> [IVIPTGUSStaSW]  "<VINP_IVIPTGUSStaSW_flg>"
  bus_selector/82 -> [USSStaFCL]  "<VOUTP_USSStaFCL_flg>"
  bus_selector/58 -> [PASAFCL]  "<VOUTP_PASAFCL_enum>"
  bus_selector/61 -> [PASDRCR]  "<VOUTP_PASDRCR_cm>"
  bus_selector/36 -> [SWCCHANCElSta]  "<VINP_SWCCANCELSta_flg>"
  bus_selector/35 -> [SWCACCsta]  "<VINP_SWCACCSta_flg>"
  bus_selector/31 -> [EpasFailed]  "<VINP_EpasFailed_enum>"
  bus_selector/28 -> [SASV]  "<VINP_SASV_flg>"
  bus_selector/16 -> [EBDActive]  "<VINP_EBDActive_flg>"
  bus_selector/12 -> [PBAActive]  "<VINP_PBAActive_flg>"
  bus_selector/22 -> [LRRawWhlSpeedV]  "<VINP_LRRawWhlSpeedV_flg>"
  bus_selector/14 -> [ABSActive]  "<VINP_ABSActive_flg>"
  bus_selector/46 -> [SWCUndefinedSta]  "<VINP_SWCUndefinedSta_flg>"
  bus_selector/77 -> [USSStaRCR]  "<VOUTP_USSStaRCR_flg>"
  bus_selector/43 -> [SWCLeftSta]  "<VINP_SWCLeftSta_flg>"
  bus_selector/73 -> [PASModOperation]  "<VOUTP_ModOperation_enum>"
  bus_selector/25 -> [LFRawWhlSpeed]  "<VINP_LFRawWhlSpeed_kph>"
  bus_selector/45 -> [SWCRegenDown]  "<VINP_SWCRegenDown_flg>"
  bus_selector/130 -> [RrTqSource]  "<VOUTP_TqSourceRr_enum>"
  bus_selector/5 -> [LatAccelV]  "<VINP_LatAccelV_flg>"
  bus_selector/76 -> [USSStaRML]  "<VOUTP_USSStaRML_flg>"
  bus_selector/33 -> [EPSTOIUnavailable]  "<VINP_EPSTOIUnavailable_flg>"
  bus_selector/128 -> [ActAPSPosn]  "<VOUTP_ActAPSPosn_pct>"
  bus_selector/23 -> [RFRawWhlSpeed]  "<VINP_RFRawWhlSpeed_kph>"
  bus_selector/91 -> [DriverDoorSwitchStatus]  "<VOUTP_DrDoorSW_flg>"
  bus_selector/44 -> [SWCRightSta]  "<VINP_SWCRightSta_flg>"
  bus_selector/30 -> [EPSAOIControl]  "<VINP_EPSAOIControl_enum>"
  bus_selector/32 -> [EPSTOIActivation]  "<VINP_EPSTOIActivation_flg>"
  bus_selector/137 -> [VTQDExtShftAllowflg]  "<VOUTP_ExtShftAllow_flg>"
  bus_selector/121 -> [LeftRearWheelTemperature]  "<VOUTP_LRWheelTemp_C>"
  bus_selector/34 -> [EPSTOIFault]  "<VINP_EPSTOIFault_flg>"
  bus_selector/7 -> [YawRateV]  "<VINP_YawRateV_flg>"
  bus_selector/59 -> [PASDRMR]  "<VOUTP_PASDRMR_cm>"
  bus_selector/51 -> [PASARMR]  "<VOUTP_PASARMR_enum>"
  bus_selector/11 -> [MCPressureV]  "<VINP_MCPressureV_flg>"
  bus_selector/17 -> [EBDFailed]  "<VINP_EBDFailed_flg>"
  bus_selector/53 -> [PASARCR]  "<VOUTP_PASARCR_enum>"
  bus_selector/40 -> [SWCmodeSta]  "<VINP_SWCmodeSta_flg>"
  bus_selector/113 -> [HVBContactorSta]  "<VINP_HVBContactorSta_flg>"
  bus_selector/10 -> [MCPressure]  "<VINP_MCPressure_bar>"
  bus_selector/41 -> [SWCUpSta]  "<VINP_SWCUpSta_flg>"
  bus_selector/8 -> [BrkSwSta]  "<VINP_BrkSwSta_flg>"
  bus_selector/21 -> [LRRawWhlSpeed]  "<VINP_LRRawWhlSpeed_kph>"
  bus_selector/26 -> [LFRawWhlSpeedV]  "<VINP_LFRawWhlSpeedV_flg>"
  bus_selector/2 -> [LongAccel]  "<VINP_LongAccel_Gps>"
  bus_selector/13 -> [PBAFailed]  "<VINP_PBAFailed_flg>"
  bus_selector/115 -> [LeftForwardWheelPressure]  "<VOUTP_LFWheelPress_raw8>"
  bus_selector/90 -> [AllDoorSwitchStatus]  "<VOUTP_AllDoorSW_flg>"
  bus_selector/24 -> [RFRawWhlSpeedV]  "<VINP_RFRawWhlSpeedV_flg>"
  bus_selector/63 -> [PASDFMR]  "<VOUTP_PASDFMR_cm>"
  bus_selector/27 -> [SASAngle]  "<VINP_SASAngle_Deg>"
  bus_selector/95 -> [TailgateSwitchStatus]  "<VOUTP_TailgateSW_flg>"
  bus_selector/93 -> [RearLeftDoorSwitchStatus]  "<VOUTP_RLDoorSW_flg>"
  bus_selector/94 -> [RearRightDoorSwitchStatus]  "<VOUTP_RRDoorSW_flg>"
  bus_selector/96 -> [HoodSwitchStatus]  "<VOUTP_HoodSW_flg>"
  bus_selector/100 -> [PositionLampStatus]  "<VOUTP_PosLamp_flg>"
  bus_selector/101 -> [LowBeamStatus]  "<VOUTP_LBeam_flg>"
  bus_selector/102 -> [HighBeamStatus]  "<VOUTP_HBeam_flg>"
  bus_selector/105 -> [LeftTurnLampStatus]  "<VOUTP_LTurnLP_flg>"
  bus_selector/106 -> [RightTurnLampStatus]  "<VOUTP_RTurnLP_flg>"
  bus_selector/107 -> [BrakeLampStatus]  "<VOUTP_BrakeLamp_flg>"
  bus_selector/108 -> [ReverseLampStatus]  "<VOUTP_ReverseLamp_flg>"
  bus_selector/109 -> [RearFogLampStatus]  "<VOUTP_RrFogLamp_flg>"
  [BOUTP_outputs] -> Bus Creator1/1  "BOUTP_outputs"
  BINP_CANx_outputs/1 -> Bus Creator1/2  "BINP_CANx_outputs"
  Bus Creator1/1 -> bus_selector/1
  UnitConverter22/1 -> SignalPack14/1
  [MCPressure] -> convert_out93/1
  [BrkSwV] -> convert_out82/1
  SignalPack16/1 -> UnitConverter26/1
  SignalPack14/1 -> UnitConverter23/1
  UnitConverter28/1 -> SignalPack18/1
  convert_out93/1 -> UnitConverter24/1
  [VTQDExtDoorAllowflg] -> convert_out137/1
  convert_out13/1 -> UnitConverter34/1
  UnitConverter53/1 -> Mux32/3
  SignalPack34/1 -> UnitConverter57/1
  SignalPack29/1 -> UnitConverter49/1
  convert_out15/1 -> UnitConverter38/1
  convert_out19/1 -> UnitConverter48/1
  [RRRawWhlSpeedV] -> convert_out19/1
  SignalPack21/1 -> UnitConverter35/1
  UnitConverter39/1 -> Mux9/9
  UnitConverter35/1 -> Mux9/7
  UnitConverter41/1 -> Mux9/10
  UnitConverter134/1 -> BitwiseAND5/2
  SignalPack79/1 -> UnitConverter140/1
  UnitConverter139/1 -> SignalPack79/1
  UnitConverter137/1 -> SignalPack78/1
  SignalPack77/1 -> UnitConverter136/1
  UnitConverter171/1 -> SignalPack95/1
  UnitConverter169/1 -> SignalPack94/1
  SignalPack94/1 -> UnitConverter170/1
  UnitConverter176/1 -> BitwiseAND6/5
  convert_out68/1 -> UnitConverter153/1
  UnitConverter154/1 -> Mux15/14
  UnitConverter165/1 -> SignalPack92/1
  UnitConverter160/1 -> Mux15/17
  UnitConverter142/1 -> Mux15/8
  convert_out14/1 -> UnitConverter36/1
  convert_out79/1 -> UnitConverter173/1
  SignalPack17/1 -> UnitConverter27/1
  SignalPack89/1 -> UnitConverter160/1
  [APSDRLR] -> convert_out70/1
  UnitConverter167/1 -> SignalPack93/1
  SignalPack92/1 -> UnitConverter166/1
  convert_out78/1 -> UnitConverter171/1
  UnitConverter151/1 -> SignalPack85/1
  SignalPack87/1 -> UnitConverter156/1
  UnitConverter170/1 -> BitwiseAND6/2
  UnitConverter136/1 -> Mux15/5
  SignalPack86/1 -> UnitConverter154/1
  convert_out72/1 -> UnitConverter159/1
  UnitConverter296/1 -> Mux30/1
  UnitConverter153/1 -> SignalPack86/1
  SignalPack53/1 -> UnitConverter88/1
  UnitConverter91/1 -> SignalPack55/1
  UnitConverter84/1 -> Mux13/7
  UnitConverter80/1 -> Mux13/5
  [EPSTOIFault] -> convert_out33/1
  [SWCACCsta] -> convert_out34/1
  [SWCCHANCElSta] -> convert_out35/1
  [SWCUpSta] -> convert_out40/1
  SignalPack39/1 -> UnitConverter64/1
  UnitConverter64/1 -> Mux10/2
  [BrkPedalPos] -> convert_out128/1
  convert_out118/1 -> UnitConverter255/1
  convert_out128/1 -> UnitConverter275/1
  UnitConverter280/1 -> SignalPack150/1, SignalPack151/1
  UnitConverter208/1 -> BitwiseAND8/8
  UnitConverter204/1 -> BitwiseAND8/6
  UnitConverter196/1 -> BitwiseAND8/2
  Mux10/1 -> Mux11/7
  Mux31/1 -> Mux11/1
  SignalPack40/1 -> UnitConverter65/1
  SignalPack44/1 -> UnitConverter71/1
  convert_out23/1 -> UnitConverter60/1
  convert_out70/1 -> UnitConverter157/1
  UnitConverter60/1 -> SignalPack37/1
  UnitConverter58/1 -> Mux33/2
  UnitConverter25/1 -> Mux8/1
  SignalPack15/1 -> UnitConverter25/1
  UnitConverter87/1 -> SignalPack53/1
  [VTQDExternalTqAllowflg] -> convert_out135/1
  [LRRawWhlSpeed] -> convert_out20/1
  convert_out135/1 -> UnitConverter295/1
  UnitConverter279/1 -> Mux29/1
  [RFRawWhlSpeed] -> convert_out22/1
  [PASARCL] -> convert_out53/1
  UnitConverter125/1 -> SignalPack72/1
  SignalPack72/1 -> UnitConverter126/1
  convert_out82/1 -> UnitConverter22/1
  SignalPack67/1 -> UnitConverter116/1
  UnitConverter116/1 -> BitwiseAND1/7
  SignalPack70/1 -> UnitConverter122/1
  UnitConverter121/1 -> SignalPack70/1
  UnitConverter122/1 -> BitwiseAND2/2
  [LVBattDet12V] -> convert_out109/1
  UnitConverter192/1 -> Mux17/1
  [IVIPTGUSStaSW] -> convert_out89/1
  SignalPack126/1 -> UnitConverter234/1
  SignalPack106/1 -> UnitConverter194/1
  UnitConverter193/1 -> SignalPack106/1
  convert_out24/1 -> UnitConverter62/1
  convert_out92/1 -> UnitConverter197/1
  convert_out110/1 -> UnitConverter239/1
  SignalPack107/1 -> UnitConverter196/1
  [HVBContactorSta] -> convert_out112/1
  Mux30/1 -> [FoxPiShifterallow]
  convert_out42/1 -> UnitConverter103/1
  [SWCLeftSta] -> convert_out42/1
  UnitConverter100/1 -> BitwiseAND/7
  UnitConverter92/1 -> BitwiseAND/3
  UnitConverter88/1 -> BitwiseAND/1
  convert_out136/1 -> UnitConverter297/1
  UnitConverter254/1 -> Mux21/4
  [ABSActive] -> convert_out13/1
  SignalPack142/1 -> UnitConverter266/1
  SignalPack141/1 -> UnitConverter264/1
  UnitConverter287/1 -> Mux26/1
  SignalPack52/1 -> UnitConverter86/1
  SignalPack38/1 -> UnitConverter63/1
  [SASCAL] -> convert_out28/1
  [EPSAOIControl] -> convert_out29/1
  convert_out27/1 -> UnitConverter73/1
  UnitConverter72/1 -> Mux12/4
  UnitConverter71/1 -> Mux12/3
  UnitConverter23/1 -> Mux9/2
  SignalPack46/1 -> UnitConverter74/1
  UnitConverter159/1 -> SignalPack89/1
  SignalPack47/1 -> UnitConverter76/1
  UnitConverter68/1 -> SignalPack45/1, SignalPack44/1, SignalPack43/1, SignalPack42/1
  UnitConverter156/1 -> Mux15/15
  UnitConverter144/1 -> Mux15/9
  convert_out53/1 -> UnitConverter125/1
  UnitConverter162/1 -> Mux15/18
  convert_out20/1 -> UnitConverter50/1
  [USSStaFCL] -> convert_out84/1
  UnitConverter166/1 -> Mux15/20
  Mux27/1 -> Mux29/5
  UnitConverter27/1 -> Mux8/3
  UnitConverter178/1 -> BitwiseAND6/6
  SignalPack90/1 -> UnitConverter162/1
  SignalPack54/1 -> UnitConverter90/1
  Mux17/1 -> [FoxPiPTGUSSSW]
  UnitConverter150/1 -> Mux15/12
  BitwiseAND4/1 -> Mux15/3
  UnitConverter161/1 -> SignalPack90/1
  convert_out77/1 -> UnitConverter169/1
  [ColumnDimSwitchStatus] -> convert_out139/1
  Mux18/1 -> [FoxPiSwitchStatus]
  convert_out101/1 -> UnitConverter221/1
  convert_out100/1 -> UnitConverter219/1
  BitwiseAND8/1 -> Mux18/1
  [HighBeamStatus] -> convert_out101/1
  [LowBeamStatus] -> convert_out100/1
  convert_out139/1 -> UnitConverter213/1
  convert_out81/1 -> UnitConverter177/1
  [USSStaFMR] -> convert_out80/1
  UnitConverter124/1 -> BitwiseAND3/1
  SignalPack71/1 -> UnitConverter124/1
  [USSStaRMR] -> convert_out76/1
  UnitConverter123/1 -> SignalPack71/1
  convert_out54/1 -> UnitConverter127/1
  [PASAFML] -> convert_out55/1
  [PASAFMR] -> convert_out54/1
  UnitConverter299/1 -> SignalPack162/1
  UnitConverter115/1 -> SignalPack67/1
  UnitConverter141/1 -> SignalPack80/1
  UnitConverter261/1 -> SignalPack140/1
  UnitConverter221/1 -> SignalPack120/1
  Mux13/1 -> [FoxPiEPSStatus]
  SignalPack138/1 -> UnitConverter258/1
  SignalPack140/1 -> UnitConverter262/1
  UnitConverter227/1 -> SignalPack123/1
  UnitConverter224/1 -> BitwiseAND9/7
  SignalPack120/1 -> UnitConverter222/1
  UnitConverter220/1 -> BitwiseAND9/5
  SignalPack62/1 -> UnitConverter106/1
  UnitConverter189/1 -> SignalPack104/1
  UnitConverter242/1 -> Mux20/3
  [SWCUndefinedSta] -> convert_out45/1
  convert_out45/1 -> UnitConverter109/1
  UnitConverter186/1 -> BitwiseAND7/2
  UnitConverter246/1 -> BitwiseAND11/2
  SignalPack108/1 -> UnitConverter198/1
  UnitConverter236/1 -> BitwiseAND10/6
  UnitConverter228/1 -> BitwiseAND10/2
  [CellTempAvg] -> convert_out111/1
  SignalPack28/1 -> UnitConverter47/1
  SignalPack23/1 -> UnitConverter39/1
  SignalPack149/1 -> UnitConverter279/1
  UnitConverter43/1 -> Mux9/11
  [ACCAvailabliity] -> convert_out17/1
  UnitConverter30/1 -> SignalPack19/1
  [PBAActive] -> convert_out11/1
  SignalPack20/1 -> UnitConverter33/1
  [SWCRightSta] -> convert_out43/1
  UnitConverter44/1 -> SignalPack27/1, SignalPack28/1, SignalPack26/1
  UnitConverter21/1 -> Mux9/1
  UnitConverter76/1 -> Mux13/3
  SignalPack31/1 -> UnitConverter52/1
  SignalPack37/1 -> UnitConverter61/1
  UnitConverter52/1 -> Mux32/2
  SignalPack36/1 -> UnitConverter59/1
  UnitConverter32/1 -> SignalPack20/1
  Mux7/1 -> [FoxPiMotionStatus]
  UnitConverter8/1 -> Mux7/3
  SignalPack12/1 -> UnitConverter19/1
  UnitConverter18/1 -> SignalPack12/1
  [SWCVRSta] -> convert_out46/1
  UnitConverter20/1 -> SignalPack13/1
  UnitConverter216/1 -> BitwiseAND9/3
  convert_out97/1 -> UnitConverter205/1
  SignalPack115/1 -> UnitConverter212/1
  [TPMSWarnindi] -> convert_out126/1
  UnitConverter300/1 -> Mux30/3
  UnitConverter31/1 -> Mux9/5
  SignalPack144/1 -> UnitConverter270/1
  UnitConverter262/1 -> Mux21/8
  UnitConverter269/1 -> SignalPack144/1
  [LFRawWhlSpeed] -> convert_out24/1
  convert_out43/1 -> UnitConverter105/1
  UnitConverter143/1 -> SignalPack81/1
  UnitConverter1/1 -> Mux3/1
  UnitConverter258/1 -> Mux21/6
  SignalPack30/1 -> UnitConverter51/1
  [PASAFCL] -> convert_out57/1
  UnitConverter157/1 -> SignalPack88/1
  convert_out98/1 -> UnitConverter207/1
  convert_out4/1 -> UnitConverter/1
  UnitConverter107/1 -> SignalPack63/1
  [Vehiclespeed] -> convert_out4/1
  UnitConverter75/1 -> SignalPack47/1
  SignalPack2/1 -> UnitConverter3/1
  [LatAccel] -> convert_out7/1
  convert_out7/1 -> UnitConverter9/1
  SignalPack158/1 -> UnitConverter293/1
  [BrkSwSta] -> convert_out71/1
  SignalPack78/1 -> UnitConverter138/1
  UnitConverter288/1 -> Mux26/2
  SignalPack48/1 -> UnitConverter78/1
  convert_out129/1 -> UnitConverter278/1
  UnitConverter29/1 -> Mux9/4
  UnitConverter277/1 -> Mux22/2
  UnitConverter3/1 -> Mux3/3
  convert_out130/1 -> UnitConverter280/1
  [RearRightDoorSwitchStatus] -> convert_out97/1
  UnitConverter6/1 -> Mux4/2
  [VTQDExtShftAllowflg] -> convert_out136/1
  [LongAccel] -> convert_out5/1
  UnitConverter4/1 -> SignalPack3/1, SignalPack4/1
  SignalPack5/1 -> UnitConverter8/1
  [PASDFCL] -> convert_out66/1
  [APSDRLL] -> convert_out69/1
  UnitConverter147/1 -> SignalPack83/1
  UnitConverter85/1 -> SignalPack52/1
  [APSDFLL] -> convert_out67/1
  convert_out73/1 -> UnitConverter161/1
  convert_out65/1 -> UnitConverter147/1
  UnitConverter36/1 -> SignalPack22/1
  [PASDFCR] -> convert_out65/1
  SignalPack84/1 -> UnitConverter150/1
  convert_out69/1 -> UnitConverter155/1
  [PASSNSRLayout] -> convert_out73/1
  convert_out94/1 -> UnitConverter199/1
  UnitConverter148/1 -> Mux15/11
  SignalPack73/1 -> UnitConverter128/1
  UnitConverter127/1 -> SignalPack73/1
  SignalPack74/1 -> UnitConverter130/1
  SignalPack42/1 -> UnitConverter69/1
  convert_out56/1 -> UnitConverter131/1
  SignalPack109/1 -> UnitConverter200/1
  SignalPack113/1 -> UnitConverter208/1
  SignalPack114/1 -> UnitConverter210/1
  UnitConverter199/1 -> SignalPack109/1
  [RightForwardWheelPressure] -> convert_out115/1
  UnitConverter295/1 -> SignalPack160/1
  SignalPack160/1 -> UnitConverter296/1
  BitwiseAND11/1 -> Mux20/4
  UnitConverter226/1 -> BitwiseAND10/1
  UnitConverter197/1 -> SignalPack108/1
  UnitConverter112/1 -> BitwiseAND1/5
  SignalPack130/1 -> UnitConverter242/1
  UnitConverter244/1 -> BitwiseAND11/1
  [USSStaFML] -> convert_out81/1
  convert_out115/1 -> UnitConverter249/1
  [SASV] -> convert_out27/1
  UnitConverter241/1 -> SignalPack130/1
  convert_out109/1 -> UnitConverter237/1
  SignalPack103/1 -> UnitConverter188/1
  UnitConverter213/1 -> SignalPack116/1
  convert_out107/1 -> UnitConverter233/1
  convert_out33/1 -> UnitConverter85/1
  [ReverseLampStatus] -> convert_out107/1
  SignalPack127/1 -> UnitConverter236/1
  convert_out57/1 -> UnitConverter133/1
  SignalPack93/1 -> UnitConverter168/1
  SignalPack102/1 -> UnitConverter186/1
  UnitConverter69/1 -> Mux12/1
  UnitConverter235/1 -> SignalPack127/1
  UnitConverter187/1 -> SignalPack103/1
  SignalPack98/1 -> UnitConverter178/1
  convert_out102/1 -> UnitConverter223/1
  SignalPack13/1 -> UnitConverter21/1
  [RightTurnLampStatus] -> convert_out105/1
  [AllDoorSwitchStatus] -> convert_out92/1
  UnitConverter298/1 -> Mux30/2
  SignalPack1/1 -> UnitConverter2/1
  UnitConverter185/1 -> SignalPack102/1
  [TailgateSwitchStatus] -> convert_out98/1
  UnitConverter177/1 -> SignalPack98/1
  [RightDaytimeRunningLightStatus] -> convert_out102/1
  convert_out84/1 -> UnitConverter181/1
  SignalPack100/1 -> UnitConverter182/1
  convert_out40/1 -> UnitConverter99/1
  [BrakeLampStatus] -> convert_out106/1
  SignalPack4/1 -> UnitConverter6/1
  convert_out83/1 -> UnitConverter179/1
  Mux11/1 -> [FoxPiWheelSpeed]
  [USSStaFCR] -> convert_out83/1
  Mux15/1 -> [FoxPiUSSDistance]
  SignalPack116/1 -> UnitConverter214/1
  UnitConverter168/1 -> BitwiseAND6/1
  convert_out39/1 -> UnitConverter97/1
  [PASDRCL] -> convert_out62/1
  convert_out62/1 -> UnitConverter141/1
  UnitConverter93/1 -> SignalPack56/1
  SignalPack19/1 -> UnitConverter31/1
  SignalPack57/1 -> UnitConverter96/1
  convert_out35/1 -> UnitConverter89/1
  Mux22/1 -> Mux23/2
  UnitConverter238/1 -> Mux20/1
  [RearLeftDoorSwitchStatus] -> convert_out96/1
  UnitConverter95/1 -> SignalPack57/1
  Mux16/1 -> [FoxPiUSSFaultStatus]
  UnitConverter130/1 -> BitwiseAND4/2
  UnitConverter138/1 -> Mux15/6
  SignalPack105/1 -> UnitConverter192/1
  UnitConverter191/1 -> SignalPack105/1
  convert_out55/1 -> UnitConverter129/1
  convert_out71/1 -> UnitConverter20/1
  convert_out91/1 -> UnitConverter195/1
  [USSStaRCR] -> convert_out78/1
  BitwiseAND6/1 -> Mux16/1
  UnitConverter188/1 -> BitwiseAND7/3
  convert_out90/1 -> UnitConverter193/1
  SignalPack58/1 -> UnitConverter98/1
  UnitConverter212/1 -> BitwiseAND9/1
  Mux28/1 -> Mux29/6
  BitwiseAND10/1 -> Mux19/2
  convert_out26/1 -> UnitConverter68/1
  SignalPack161/1 -> UnitConverter298/1
  SignalPack45/1 -> UnitConverter72/1
  UnitConverter49/1 -> Mux11/2
  UnitConverter260/1 -> Mux21/7
  UnitConverter66/1 -> SignalPack41/1
  convert_out140/1 -> UnitConverter215/1
  UnitConverter55/1 -> Mux11/4
  SignalPack85/1 -> UnitConverter152/1
  convert_out25/1 -> UnitConverter66/1
  [LFRawWhlSpeedV] -> convert_out25/1
  UnitConverter65/1 -> Mux10/3
  UnitConverter63/1 -> Mux10/1
  SignalPack43/1 -> UnitConverter70/1
  Mux23/1 -> [FoxPiPedalposition]
  SignalPack55/1 -> UnitConverter92/1
  [SWCRegenDown] -> convert_out44/1
  Mux25/1 -> Mux29/3
  [TMSpd] -> convert_out134/1
  UnitConverter294/1 -> Mux28/2
  UnitConverter195/1 -> SignalPack107/1
  UnitConverter14/1 -> SignalPack10/1, SignalPack11/1, SignalPack9/1
  UnitConverter42/1 -> SignalPack25/1
  UnitConverter37/1 -> Mux9/8
  convert_out89/1 -> UnitConverter191/1
  UnitConverter33/1 -> Mux9/6
  Mux9/1 -> [FoxPiBrakeStatus]
  convert_out21/1 -> UnitConverter54/1
  convert_out12/1 -> UnitConverter32/1
  convert_out18/1 -> UnitConverter44/1
  Mux6/1 -> Mux7/6
  UnitConverter46/1 -> Mux31/2
  convert_out34/1 -> UnitConverter87/1
  UnitConverter16/1 -> Mux6/2
  SignalPack33/1 -> UnitConverter55/1
  UnitConverter70/1 -> Mux12/2
  SignalPack27/1 -> UnitConverter46/1
  [APSDFLR] -> convert_out68/1
  UnitConverter54/1 -> SignalPack33/1
  UnitConverter225/1 -> SignalPack122/1
  UnitConverter19/1 -> Mux7/7
  UnitConverter145/1 -> SignalPack82/1
  UnitConverter181/1 -> SignalPack100/1
  SignalPack26/1 -> UnitConverter45/1
  UnitConverter284/1 -> Mux25/1
  UnitConverter73/1 -> SignalPack46/1
  [SWCmodeSta] -> convert_out39/1
  UnitConverter283/1 -> SignalPack152/1, SignalPack153/1
  convert_out37/1 -> UnitConverter93/1
  UnitConverter50/1 -> SignalPack31/1, SignalPack32/1, SignalPack30/1
  SignalPack41/1 -> UnitConverter67/1
  convert_out67/1 -> UnitConverter151/1
  UnitConverter103/1 -> SignalPack61/1
  UnitConverter102/1 -> BitwiseAND/8
  BitwiseAND3/1 -> Mux15/2
  UnitConverter98/1 -> BitwiseAND/6
  convert_out41/1 -> UnitConverter101/1
  UnitConverter59/1 -> Mux33/3
  UnitConverter90/1 -> BitwiseAND/2
  convert_out48/1 -> UnitConverter115/1
  UnitConverter97/1 -> SignalPack58/1
  SignalPack64/1 -> UnitConverter110/1
  UnitConverter273/1 -> SignalPack146/1
  SignalPack61/1 -> UnitConverter104/1
  UnitConverter209/1 -> SignalPack114/1
  UnitConverter109/1 -> SignalPack64/1
  [PositionLampStatus] -> convert_out141/1
  convert_out104/1 -> UnitConverter227/1
  [RightRearWheelPressure] -> convert_out117/1
  SignalPack137/1 -> UnitConverter256/1
  UnitConverter180/1 -> BitwiseAND6/7
  UnitConverter255/1 -> SignalPack137/1
  UnitConverter131/1 -> SignalPack75/1
  [RFRawWhlSpeedV] -> convert_out23/1
  UnitConverter214/1 -> BitwiseAND9/2
  UnitConverter57/1 -> Mux33/1
  [LeftTurnLampStatus] -> convert_out104/1
  [LeftDaytimeRunningLightStatus] -> convert_out103/1
  convert_out76/1 -> UnitConverter167/1
  [SWCRESupSta] -> convert_out37/1
  SignalPack119/1 -> UnitConverter220/1
  [CrashDetectStatus] -> convert_out90/1
  SignalPack81/1 -> UnitConverter144/1
  UnitConverter240/1 -> Mux20/2
  convert_out141/1 -> UnitConverter217/1
  convert_out29/1 -> UnitConverter77/1
  UnitConverter219/1 -> SignalPack119/1
  SignalPack24/1 -> UnitConverter41/1
  convert_out117/1 -> UnitConverter253/1
  [ColumnTurnlampSwitchStatus] -> convert_out138/1
  UnitConverter24/1 -> SignalPack16/1, SignalPack17/1, SignalPack15/1
  UnitConverter51/1 -> Mux32/1
  UnitConverter217/1 -> SignalPack118/1
  UnitConverter174/1 -> BitwiseAND6/4
  SignalPack118/1 -> UnitConverter218/1
  [LeftForwardWheelTemperature] -> convert_out118/1
  convert_out99/1 -> UnitConverter209/1
  SignalPack117/1 -> UnitConverter216/1
  UnitConverter215/1 -> SignalPack117/1
  SignalPack112/1 -> UnitConverter206/1
  [RrTqSource] -> convert_out129/1
  UnitConverter38/1 -> SignalPack23/1
  [HoodSwitchStatus] -> convert_out99/1
  SignalPack110/1 -> UnitConverter202/1
  [SASAngle] -> convert_out26/1
  UnitConverter202/1 -> BitwiseAND8/5
  UnitConverter205/1 -> SignalPack112/1
  convert_out46/1 -> UnitConverter111/1
  convert_out9/1 -> UnitConverter14/1
  Mux14/1 -> [FoxPiButtonStatus]
  UnitConverter126/1 -> BitwiseAND3/2
  UnitConverter222/1 -> BitwiseAND9/6
  SignalPack10/1 -> UnitConverter16/1
  convert_out134/1 -> UnitConverter292/1
  SignalPack35/1 -> UnitConverter58/1
  convert_out8/1 -> UnitConverter12/1
  convert_out126/1 -> UnitConverter271/1
  [YawRate] -> convert_out9/1
  UnitConverter266/1 -> Mux21/10
  UnitConverter12/1 -> SignalPack8/1
  SignalPack104/1 -> UnitConverter190/1
  SignalPack7/1 -> UnitConverter11/1
  UnitConverter265/1 -> SignalPack142/1
  convert_out28/1 -> UnitConverter75/1
  UnitConverter274/1 -> Mux23/1
  SignalPack6/1 -> UnitConverter10/1
  SignalPack82/1 -> UnitConverter146/1
  convert_out60/1 -> UnitConverter18/1
  convert_out10/1 -> UnitConverter28/1
  UnitConverter5/1 -> Mux4/1
  convert_out96/1 -> UnitConverter203/1
  [MCPressureV] -> convert_out10/1
  [USSStaRML] -> convert_out77/1
  UnitConverter15/1 -> Mux6/1
  convert_out138/1 -> UnitConverter211/1
  convert_out112/1 -> UnitConverter243/1
  UnitConverter17/1 -> Mux6/3
  UnitConverter56/1 -> SignalPack35/1, SignalPack36/1, SignalPack34/1
  SignalPack9/1 -> UnitConverter15/1
  SignalPack80/1 -> UnitConverter142/1
  SignalPack146/1 -> UnitConverter274/1
  SignalPack11/1 -> UnitConverter17/1
  UnitConverter281/1 -> Mux24/1
  convert_out122/1 -> UnitConverter263/1
  convert_out125/1 -> UnitConverter269/1
  SignalPack8/1 -> UnitConverter13/1
  [PBAFailed] -> convert_out12/1
  [RightRearLowPressureThreshold] -> convert_out125/1
  convert_out120/1 -> UnitConverter259/1
  UnitConverter211/1 -> SignalPack115/1
  UnitConverter67/1 -> Mux11/8
  convert_out124/1 -> UnitConverter267/1
  [EBDFailed] -> convert_out16/1
  UnitConverter278/1 -> SignalPack149/1
  SignalPack25/1 -> UnitConverter43/1
  [RightRearWheelTemperature] -> convert_out121/1
  SignalPack22/1 -> UnitConverter37/1
  convert_out127/1 -> UnitConverter273/1
  UnitConverter267/1 -> SignalPack143/1
  SignalPack63/1 -> UnitConverter108/1
  UnitConverter101/1 -> SignalPack60/1
  [ActAPSPosn] -> convert_out127/1
  [LeftRearLowPressureThreshold] -> convert_out124/1
  UnitConverter290/1 -> Mux27/1
  UnitConverter182/1 -> BitwiseAND6/8
  SignalPack101/1 -> UnitConverter184/1
  convert_out87/1 -> UnitConverter187/1
  SignalPack32/1 -> UnitConverter53/1
  [USSStaFLL] -> convert_out88/1
  convert_out103/1 -> UnitConverter225/1
  convert_out88/1 -> UnitConverter189/1
  UnitConverter183/1 -> SignalPack101/1
  UnitConverter135/1 -> SignalPack77/1
  UnitConverter10/1 -> Mux5/1
  UnitConverter128/1 -> BitwiseAND4/1
  SignalPack123/1 -> UnitConverter228/1
  [RrMotorAvailTq] -> convert_out132/1
  [SWCDistanceSta] -> convert_out38/1
  UnitConverter264/1 -> Mux21/9
  UnitConverter276/1 -> Mux22/1
  [PASARCR] -> convert_out52/1
  convert_out50/1 -> UnitConverter119/1
  UnitConverter11/1 -> Mux5/2
  SignalPack68/1 -> UnitConverter118/1
  UnitConverter117/1 -> SignalPack68/1
  [PASARML] -> convert_out51/1
  [LatAccelV] -> convert_out8/1
  BitwiseAND1/1 -> Mux14/2
  convert_out52/1 -> UnitConverter123/1
  [PASDFMR] -> convert_out63/1
  [ColumnPassSwitchStatus] -> convert_out140/1
  convert_out49/1 -> UnitConverter117/1
  UnitConverter26/1 -> Mux8/2
  UnitConverter114/1 -> BitwiseAND1/6
  convert_out80/1 -> UnitConverter175/1
  SignalPack76/1 -> UnitConverter134/1
  UnitConverter203/1 -> SignalPack111/1
  UnitConverter106/1 -> BitwiseAND1/2
  UnitConverter118/1 -> BitwiseAND1/8
  Mux3/1 -> Mux7/1
  UnitConverter194/1 -> BitwiseAND8/1
  UnitConverter110/1 -> BitwiseAND1/4
  SignalPack60/1 -> UnitConverter102/1
  [SWCTripSta] -> convert_out49/1
  UnitConverter120/1 -> BitwiseAND2/1
  convert_out51/1 -> UnitConverter121/1
  SignalPack88/1 -> UnitConverter158/1
  [PASDRCR] -> convert_out61/1
  UnitConverter7/1 -> SignalPack5/1
  UnitConverter223/1 -> SignalPack121/1
  convert_out58/1 -> UnitConverter135/1
  [PASDRMR] -> convert_out58/1
  UnitConverter198/1 -> BitwiseAND8/3
  UnitConverter252/1 -> Mux21/3
  convert_out6/1 -> UnitConverter7/1
  UnitConverter132/1 -> BitwiseAND5/1
  SignalPack66/1 -> UnitConverter114/1
  convert_out61/1 -> UnitConverter139/1
  UnitConverter263/1 -> SignalPack141/1
  Mux12/1 -> Mux13/1
  UnitConverter13/1 -> Mux7/5
  convert_out59/1 -> UnitConverter137/1
  convert_out11/1 -> UnitConverter30/1
  [EBDActive] -> convert_out15/1
  UnitConverter270/1 -> Mux21/12
  convert_out137/1 -> UnitConverter299/1
  SignalPack59/1 -> UnitConverter100/1
  SignalPack148/1 -> UnitConverter277/1
  [LongAccelV] -> convert_out6/1
  UnitConverter259/1 -> SignalPack139/1
  UnitConverter77/1 -> SignalPack48/1
  convert_out17/1 -> UnitConverter42/1
  BitwiseAND7/1 -> Mux16/2
  [RightForwardWheelTemperature] -> convert_out119/1
  SignalPack135/1 -> UnitConverter252/1
  UnitConverter251/1 -> SignalPack135/1
  convert_out132/1 -> UnitConverter286/1
  convert_out123/1 -> UnitConverter265/1
  convert_out16/1 -> UnitConverter40/1
  SignalPack75/1 -> UnitConverter132/1
  UnitConverter172/1 -> BitwiseAND6/3
  UnitConverter271/1 -> SignalPack145/1
  convert_out95/1 -> UnitConverter201/1
  [USSStaFLR] -> convert_out87/1
  SignalPack145/1 -> UnitConverter272/1
  SignalPack162/1 -> UnitConverter300/1
  convert_out116/1 -> UnitConverter251/1
  [RightForwardLowPressureThreshold] -> convert_out123/1
  convert_out113/1 -> UnitConverter245/1
  [ABSFailed] -> convert_out14/1
  [RrTMTqReqtoNidec] -> convert_out130/1
  SignalPack/1 -> UnitConverter1/1
  SignalPack139/1 -> UnitConverter260/1
  [DriverDoorSwitchStatus] -> convert_out94/1
  [SWCRegenUp] -> convert_out48/1
  [LeftRearWheelPressure] -> convert_out116/1
  [SWCDownSta] -> convert_out41/1
  UnitConverter245/1 -> SignalPack132/1
  [LRRawWhlSpeedV] -> convert_out21/1
  UnitConverter133/1 -> SignalPack76/1
  SignalPack132/1 -> UnitConverter246/1
  UnitConverter248/1 -> Mux21/1
  SignalPack134/1 -> UnitConverter250/1
  Mux8/1 -> Mux9/3
  [PassengerDoorSwitchStatus] -> convert_out95/1
  UnitConverter247/1 -> SignalPack133/1
  SignalPack133/1 -> UnitConverter248/1
  UnitConverter249/1 -> SignalPack134/1
  Mux20/1 -> [FoxPiBatteryStatus]
  SignalPack65/1 -> UnitConverter112/1
  [SWCLKASta] -> convert_out47/1
  SignalPack69/1 -> UnitConverter120/1
  convert_out66/1 -> UnitConverter149/1
  UnitConverter119/1 -> SignalPack69/1
  convert_out47/1 -> UnitConverter113/1
  UnitConverter104/1 -> BitwiseAND1/1
  UnitConverter243/1 -> SignalPack131/1
  SignalPack56/1 -> UnitConverter94/1
  SignalPack124/1 -> UnitConverter230/1
  UnitConverter231/1 -> SignalPack125/1
  convert_out119/1 -> UnitConverter257/1
  BitwiseAND9/1 -> Mux19/1
  SignalPack122/1 -> UnitConverter226/1
  [USSStaRCL] -> convert_out79/1
  UnitConverter94/1 -> BitwiseAND/4
  UnitConverter234/1 -> BitwiseAND10/5
  SignalPack129/1 -> UnitConverter240/1
  UnitConverter229/1 -> SignalPack124/1
  SignalPack147/1 -> UnitConverter276/1
  UnitConverter/1 -> SignalPack1/1, SignalPack2/1, SignalPack/1
  SignalPack136/1 -> UnitConverter254/1
  SignalPack121/1 -> UnitConverter224/1
  SignalPack131/1 -> UnitConverter244/1
  UnitConverter149/1 -> SignalPack84/1
  UnitConverter253/1 -> SignalPack136/1
  UnitConverter111/1 -> SignalPack65/1
  convert_out108/1 -> UnitConverter235/1
  [LeftRearWheelTemperature] -> convert_out120/1
  SignalPack128/1 -> UnitConverter238/1
  UnitConverter239/1 -> SignalPack129/1
  UnitConverter62/1 -> SignalPack39/1, SignalPack40/1, SignalPack38/1
  UnitConverter237/1 -> SignalPack128/1
  [RearFogLampStatus] -> convert_out108/1
  Mux21/1 -> [FoxPiTPMSStatus]
  UnitConverter291/1 -> Mux27/2
  UnitConverter289/1 -> SignalPack156/1, SignalPack157/1
  UnitConverter99/1 -> SignalPack59/1
  [PASAFCR] -> convert_out56/1
  SignalPack83/1 -> UnitConverter148/1
  UnitConverter286/1 -> SignalPack154/1, SignalPack155/1
  UnitConverter201/1 -> SignalPack110/1
  Mux4/1 -> Mux7/2
  SignalPack97/1 -> UnitConverter176/1
  UnitConverter48/1 -> SignalPack29/1
  convert_out75/1 -> UnitConverter165/1
  UnitConverter230/1 -> BitwiseAND10/3
  UnitConverter164/1 -> Mux15/19
  UnitConverter96/1 -> BitwiseAND/5
  SignalPack111/1 -> UnitConverter204/1
  convert_out86/1 -> UnitConverter185/1
  [DriverLockStatus] -> convert_out91/1
  SignalPack91/1 -> UnitConverter164/1
  UnitConverter146/1 -> Mux15/10
  UnitConverter2/1 -> Mux3/2
  UnitConverter275/1 -> SignalPack147/1, SignalPack148/1
  UnitConverter210/1 -> Mux18/2
  UnitConverter173/1 -> SignalPack96/1
  UnitConverter45/1 -> Mux31/1
  [USSStaRLL] -> convert_out86/1
  UnitConverter113/1 -> SignalPack66/1
  UnitConverter129/1 -> SignalPack74/1
  [PASStaFSys] -> convert_out75/1
  UnitConverter218/1 -> BitwiseAND9/4
  SignalPack49/1 -> UnitConverter80/1
  UnitConverter40/1 -> SignalPack24/1
  UnitConverter86/1 -> Mux13/8
  SignalPack99/1 -> UnitConverter180/1
  convert_out5/1 -> UnitConverter4/1
  UnitConverter184/1 -> BitwiseAND7/1
  [RRRawWhlSpeed] -> convert_out18/1
  [PASModOperation] -> convert_out74/1
  UnitConverter82/1 -> Mux13/6
  SignalPack50/1 -> UnitConverter82/1
  UnitConverter155/1 -> SignalPack87/1
  convert_out74/1 -> UnitConverter163/1
  UnitConverter297/1 -> SignalPack161/1
  [EPSTOIActivation] -> convert_out31/1
  UnitConverter47/1 -> Mux31/3
  convert_out36/1 -> UnitConverter91/1
  [HVBattErr] -> convert_out113/1
  UnitConverter152/1 -> Mux15/13
  UnitConverter200/1 -> BitwiseAND8/4
  convert_out30/1 -> UnitConverter79/1
  UnitConverter83/1 -> SignalPack51/1
  UnitConverter233/1 -> SignalPack126/1
  SignalPack125/1 -> UnitConverter232/1
  UnitConverter61/1 -> Mux11/6
  SignalPack3/1 -> UnitConverter5/1
  UnitConverter268/1 -> Mux21/11
  UnitConverter175/1 -> SignalPack97/1
  convert_out38/1 -> UnitConverter95/1
  [EPSTOIUnavailable] -> convert_out32/1
  convert_out64/1 -> UnitConverter145/1
  UnitConverter81/1 -> SignalPack50/1
  convert_out63/1 -> UnitConverter143/1
  UnitConverter272/1 -> Mux21/13
  [PASChime] -> convert_out72/1
  UnitConverter232/1 -> BitwiseAND10/4
  SignalPack155/1 -> UnitConverter288/1
  [PASDRML] -> convert_out59/1
  UnitConverter293/1 -> Mux28/1
  BitwiseAND/1 -> Mux14/1
  [SWCSETdownSta] -> convert_out36/1
  UnitConverter250/1 -> Mux21/2
  UnitConverter108/1 -> BitwiseAND1/3
  convert_out131/1 -> UnitConverter283/1
  UnitConverter158/1 -> Mux15/16
  SignalPack143/1 -> UnitConverter268/1
  UnitConverter256/1 -> Mux21/5
  UnitConverter9/1 -> SignalPack6/1, SignalPack7/1
  convert_out121/1 -> UnitConverter261/1
  [RrEDURealTMTqNidec] -> convert_out131/1
  UnitConverter179/1 -> SignalPack99/1
  UnitConverter282/1 -> Mux24/2
  SignalPack51/1 -> UnitConverter84/1
  SignalPack156/1 -> UnitConverter290/1
  UnitConverter163/1 -> SignalPack91/1
  convert_out44/1 -> UnitConverter107/1
  [HVBattSOC] -> convert_out110/1
  convert_out133/1 -> UnitConverter289/1
  SignalPack95/1 -> UnitConverter172/1
  [PASDFML] -> convert_out64/1
  UnitConverter257/1 -> SignalPack138/1
  convert_out111/1 -> UnitConverter241/1
  UnitConverter78/1 -> Mux13/4
  UnitConverter140/1 -> Mux15/7
  SignalPack18/1 -> UnitConverter29/1
  Mux33/1 -> Mux11/5
  convert_out31/1 -> UnitConverter81/1
  [LeftForwardWheelPressure] -> convert_out114/1
  [RrRegenAvailTq] -> convert_out133/1
  UnitConverter105/1 -> SignalPack62/1
  UnitConverter34/1 -> SignalPack21/1
  UnitConverter74/1 -> Mux13/2
  Mux24/1 -> Mux29/2
  SignalPack154/1 -> UnitConverter287/1
  UnitConverter207/1 -> SignalPack113/1
  convert_out22/1 -> UnitConverter56/1
  SignalPack150/1 -> UnitConverter281/1
  convert_out114/1 -> UnitConverter247/1
  UnitConverter79/1 -> SignalPack49/1
  [YawRateV] -> convert_out60/1
  BitwiseAND2/1 -> Mux15/1
  SignalPack153/1 -> UnitConverter285/1
  SignalPack96/1 -> UnitConverter174/1
  SignalPack152/1 -> UnitConverter284/1
  UnitConverter190/1 -> BitwiseAND7/4
  [LeftForwardLowPressureThreshold] -> convert_out122/1
  [EpasFailed] -> convert_out30/1
  Mux29/1 -> [FoxPiMotorStatus]
  convert_out32/1 -> UnitConverter83/1
  Mux26/1 -> Mux29/4
  UnitConverter89/1 -> SignalPack54/1
  Mux5/1 -> Mux7/4
  [PASARMR] -> convert_out50/1
  SignalPack157/1 -> UnitConverter291/1
  UnitConverter206/1 -> BitwiseAND8/7
  [USSStaRLR] -> convert_out85/1
  convert_out106/1 -> UnitConverter231/1
  SignalPack151/1 -> UnitConverter282/1
  BitwiseAND5/1 -> Mux15/4
  Mux19/1 -> [FoxPiLampStatus]
  UnitConverter292/1 -> SignalPack158/1, SignalPack159/1
  convert_out105/1 -> UnitConverter229/1
  convert_out85/1 -> UnitConverter183/1
  UnitConverter285/1 -> Mux25/2
  Mux32/1 -> Mux11/3
  SignalPack159/1 -> UnitConverter294/1
  bus_selector/37 -> [SWCSETdownSta]  "<VINP_SWCSetdownSta_flg>"
  bus_selector/42 -> [SWCDownSta]  "<VINP_SWCDownSta_flg>"
  bus_selector/124 -> [RightForwardLowPressureThreshold]  "<VOUTP_RFWheelPSW_raw8>"
  bus_selector/125 -> [LeftRearLowPressureThreshold]  "<VOUTP_LRWheelPSW_raw8>"
